simulink model "D_20231120_Modell_Inbetriebnahme_BreakOutBox_Jetson"  (R2022b)
settings: Solver=ode1  StartTime=0.0  StopTime=inf  FixedStep=Ts  RelTol=1e-3
PreLoadFcn:
  | pulsePeriod = 0.05;
  | 
  | Ts = 0.001;
  | 
  | FPGA_Frequency = 75000000;
  | 
  | ts_IO691 = 5e-3;
PostLoadFcn:
  | ewolfSetUp
InitFcn:
  | pulsePeriod = 0.05;
  | 
  | Ts = 0.001;
  | 
  | FPGA_Frequency = 75000000;
  | 
  | ts_IO691 = 5e-3;
StopFcn:
  | Simulink.sdi.clearPreferences;
  | if isfile(['sdi_view_',bdroot,'.mldatx'])
  | Simulink.sdi.view;
  | pause(3);
  | Simulink.sdi.loadView(['sdi_view_',bdroot,]);
  | end
model workspace (MAT data in the model file):
  MaxDreh = 1
values from neighbouring files (symbols this model uses):
  max_ac = 2    [ewolfSetUp.m]
  min_ac = -3    [ewolfSetUp.m]
  PredictionHorizon = 30    [ewolfSetUp.m]
undefined symbols (not defined in the file or in its folder): canChannel, DiscIntNeverNeededParam, Ended, HS, IO291, IO397, max_steer_car, min_steer_car, sigbuilder_block, Single
libraries: lllalib x255, canmsglib x146, simulink x42, speedgoatlib_IO191 x5, speedgoatlib_IO291 x5, slrealtimeiplib x3, speedgoatlib_IO691 x3, slrealtimeutilitieslib x2, spsEdgeDetectorLib x1, simulink_extras x1, speedgoatlib_fpga_dio x1, speedgoatlib_fpga_quadrature x1
(part 4 of 8)

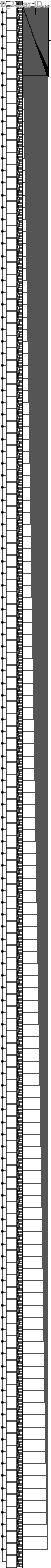
== system D_20231120_Modell_Inbetriebnahme_BreakOutBox_Jetson/IO691/CAN Read Loop - Port 3/Radar IDs einlesen (128) ==
  CAN Msg : Inport
  Bus Creator : BusCreator  Inputs=5
  Bus Creator1 : BusCreator  Inputs=129
  Bus Creator{2..129} (128 alike) : BusCreator  Inputs=8
  CAN Unpack1 : canmsglib/CAN Unpack  CANdbFile=eWolf_SensorCAN.dbc  MsgList=Radar_Sensor_Control  MsgName=Radar_Sensor_Control  MsgIDType=Standard (11-bit identifier)  MsgIdentifier=1024  MsgLength=8  SignalInfo={'Cycle_Duration','0','12','LE','unsigned','Standard','0','0.064','0','0','262';'Cycle_counter','15','32','LE','unsigned','Standard','0','1','0','-Inf','Inf';'Number_of_Objects','47','8','LE','unsigned','Standard','0','1','0','0','255';'Reserve','12','3','LE','unsigned','Standard','0','1','0','-Inf','Inf';'Reserve_2','55','9','LE','unsigned','Standard','0','1','0','-Inf','Inf'}  IDPort=on  TimestampPort=on  ErrorPort=off  RemotePort=off  LengthPort=off  StatusPort=off  ApplyMinMax=off
      settings: DataFormat=CANdb specified signals
  CAN Unpack10 : canmsglib/CAN Unpack  CANdbFile=eWolf_SensorCAN.dbc  MsgList=Radar_RawTarget_Data_009  MsgName=Radar_RawTarget_Data_009  MsgIDType=Standard (11-bit identifier)  MsgIdentifier=1033  MsgLength=8  SignalInfo={'AZ_Winkel','22','10','LE','unsigned','Multiplexed','0','0.16','-81.76','-81.76','81.92';'EL_Angle','37','10','LE','unsigned','Multiplexed','1','0.04','-20.44','-20.44','20.48';'Internal_used','14','8','LE','unsigned','Multiplexed','0','1','0','-Inf','Inf';'Internal_used2','32','7','LE','unsigned','Multiplexed','0','1','0','-Inf','Inf';'Internal_used3','51','7','LE','unsigned','Multiplexed','0','1','0','-Inf','Inf';'Internal_used4','58','6','LE','unsigned','Multiplexed','0','1','0','-Inf','Inf';'Internal_used5','9','8','LE','unsigned','Multiplexed','1','1','0','-Inf','Inf';'Internal_used6','17','8','LE','unsigned','Multiplexed','1','1','0','-Inf','Inf';'Internal_used7','25','7','LE','unsigned','Multiplexed','1','1','0','-Inf','Inf';'Mode_Signal','0','1','LE','unsigned','Multiplexor','0','1','0','0','1';'RCS','1','7','LE','unsigned','Multiplexed','1','0.2','-15','-15','36';'Range1','1','13','LE','unsigned','Multiplexed','0','0.04','0','0','327.64';'Reserve_3','32','5','LE','unsigned','Multiplexed','1','1','0','-Inf','Inf';'Reserve_4','47','16','LE','unsigned','Multiplexed','1','1','0','-Inf','Inf';'Speed_Radial','39','12','LE','unsigned','Multiplexed','0','0.04','-119.68','-44.12','119.68'}  IDPort=on  TimestampPort=on  ErrorPort=off  RemotePort=off  LengthPort=off  StatusPort=off  ApplyMinMax=off
      settings: DataFormat=CANdb specified signals
  CAN Unpack100 : canmsglib/CAN Unpack  CANdbFile=eWolf_SensorCAN.dbc  MsgList=Radar_RawTarget_Data_099  MsgName=Radar_RawTarget_Data_099  MsgIDType=Standard (11-bit identifier)  MsgIdentifier=1123  MsgLength=8  SignalInfo={'AZ_Winkel','22','10','LE','unsigned','Multiplexed','0','0.16','-81.76','-81.76','81.92';'EL_Angle','37','10','LE','unsigned','Multiplexed','1','0.04','-20.44','-20.44','20.48';'Internal_used','14','8','LE','unsigned','Multiplexed','0','1','0','-Inf','Inf';'Internal_used2','32','7','LE','unsigned','Multiplexed','0','1','0','-Inf','Inf';'Internal_used3','51','7','LE','unsigned','Multiplexed','0','1','0','-Inf','Inf';'Internal_used4','58','6','LE','unsigned','Multiplexed','0','1','0','-Inf','Inf';'Internal_used5','9','8','LE','unsigned','Multiplexed','1','1','0','-Inf','Inf';'Internal_used6','17','8','LE','unsigned','Multiplexed','1','1','0','-Inf','Inf';'Internal_used7','25','7','LE','unsigned','Multiplexed','1','1','0','-Inf','Inf';'Mode_Signal','0','1','LE','unsigned','Multiplexor','0','1','0','0','1';'RCS','1','7','LE','unsigned','Multiplexed','1','0.2','-15','-15','36';'Range1','1','13','LE','unsigned','Multiplexed','0','0.04','0','0','327.64';'Reserve_3','32','5','LE','unsigned','Multiplexed','1','1','0','-Inf','Inf';'Reserve_4','47','16','LE','unsigned','Multiplexed','1','1','0','-Inf','Inf';'Speed_Radial','39','12','LE','unsigned','Multiplexed','0','0.04','-119.68','-44.12','119.68'}  IDPort=on  TimestampPort=on  ErrorPort=off  RemotePort=off  LengthPort=off  StatusPort=off  ApplyMinMax=off
      settings: DataFormat=CANdb specified signals
  CAN Unpack101 : canmsglib/CAN Unpack  CANdbFile=eWolf_SensorCAN.dbc  MsgList=Radar_RawTarget_Data_100  MsgName=Radar_RawTarget_Data_100  MsgIDType=Standard (11-bit identifier)  MsgIdentifier=1124  MsgLength=8  SignalInfo={'AZ_Winkel','22','10','LE','unsigned','Multiplexed','0','0.16','-81.76','-81.76','81.92';'EL_Angle','37','10','LE','unsigned','Multiplexed','1','0.04','-20.44','-20.44','20.48';'Internal_used','14','8','LE','unsigned','Multiplexed','0','1','0','-Inf','Inf';'Internal_used2','32','7','LE','unsigned','Multiplexed','0','1','0','-Inf','Inf';'Internal_used3','51','7','LE','unsigned','Multiplexed','0','1','0','-Inf','Inf';'Internal_used4','58','6','LE','unsigned','Multiplexed','0','1','0','-Inf','Inf';'Internal_used5','9','8','LE','unsigned','Multiplexed','1','1','0','-Inf','Inf';'Internal_used6','17','8','LE','unsigned','Multiplexed','1','1','0','-Inf','Inf';'Internal_used7','25','7','LE','unsigned','Multiplexed','1','1','0','-Inf','Inf';'Mode_Signal','0','1','LE','unsigned','Multiplexor','0','1','0','0','1';'RCS','1','7','LE','unsigned','Multiplexed','1','0.2','-15','-15','36';'Range1','1','13','LE','unsigned','Multiplexed','0','0.04','0','0','327.64';'Reserve_3','32','5','LE','unsigned','Multiplexed','1','1','0','-Inf','Inf';'Reserve_4','47','16','LE','unsigned','Multiplexed','1','1','0','-Inf','Inf';'Speed_Radial','39','12','LE','unsigned','Multiplexed','0','0.04','-119.68','-44.12','119.68'}  IDPort=on  TimestampPort=on  ErrorPort=off  RemotePort=off  LengthPort=off  StatusPort=off  ApplyMinMax=off
      settings: DataFormat=CANdb specified signals
  CAN Unpack102 : canmsglib/CAN Unpack  CANdbFile=eWolf_SensorCAN.dbc  MsgList=Radar_RawTarget_Data_101  MsgName=Radar_RawTarget_Data_101  MsgIDType=Standard (11-bit identifier)  MsgIdentifier=1125  MsgLength=8  SignalInfo={'AZ_Winkel','22','10','LE','unsigned','Multiplexed','0','0.16','-81.76','-81.76','81.92';'EL_Angle','37','10','LE','unsigned','Multiplexed','1','0.04','-20.44','-20.44','20.48';'Internal_used','14','8','LE','unsigned','Multiplexed','0','1','0','-Inf','Inf';'Internal_used2','32','7','LE','unsigned','Multiplexed','0','1','0','-Inf','Inf';'Internal_used3','51','7','LE','unsigned','Multiplexed','0','1','0','-Inf','Inf';'Internal_used4','58','6','LE','unsigned','Multiplexed','0','1','0','-Inf','Inf';'Internal_used5','9','8','LE','unsigned','Multiplexed','1','1','0','-Inf','Inf';'Internal_used6','17','8','LE','unsigned','Multiplexed','1','1','0','-Inf','Inf';'Internal_used7','25','7','LE','unsigned','Multiplexed','1','1','0','-Inf','Inf';'Mode_Signal','0','1','LE','unsigned','Multiplexor','0','1','0','0','1';'RCS','1','7','LE','unsigned','Multiplexed','1','0.2','-15','-15','36';'Range1','1','13','LE','unsigned','Multiplexed','0','0.04','0','0','327.64';'Reserve_3','32','5','LE','unsigned','Multiplexed','1','1','0','-Inf','Inf';'Reserve_4','47','16','LE','unsigned','Multiplexed','1','1','0','-Inf','Inf';'Speed_Radial','39','12','LE','unsigned','Multiplexed','0','0.04','-119.68','-44.12','119.68'}  IDPort=on  TimestampPort=on  ErrorPort=off  RemotePort=off  LengthPort=off  StatusPort=off  ApplyMinMax=off
      settings: DataFormat=CANdb specified signals
  CAN Unpack103 : canmsglib/CAN Unpack  CANdbFile=eWolf_SensorCAN.dbc  MsgList=Radar_RawTarget_Data_102  MsgName=Radar_RawTarget_Data_102  MsgIDType=Standard (11-bit identifier)  MsgIdentifier=1126  MsgLength=8  SignalInfo={'AZ_Winkel','22','10','LE','unsigned','Multiplexed','0','0.16','-81.76','-81.76','81.92';'EL_Angle','37','10','LE','unsigned','Multiplexed','1','0.04','-20.44','-20.44','20.48';'Internal_used','14','8','LE','unsigned','Multiplexed','0','1','0','-Inf','Inf';'Internal_used2','32','7','LE','unsigned','Multiplexed','0','1','0','-Inf','Inf';'Internal_used3','51','7','LE','unsigned','Multiplexed','0','1','0','-Inf','Inf';'Internal_used4','58','6','LE','unsigned','Multiplexed','0','1','0','-Inf','Inf';'Internal_used5','9','8','LE','unsigned','Multiplexed','1','1','0','-Inf','Inf';'Internal_used6','17','8','LE','unsigned','Multiplexed','1','1','0','-Inf','Inf';'Internal_used7','25','7','LE','unsigned','Multiplexed','1','1','0','-Inf','Inf';'Mode_Signal','0','1','LE','unsigned','Multiplexor','0','1','0','0','1';'RCS','1','7','LE','unsigned','Multiplexed','1','0.2','-15','-15','36';'Range1','1','13','LE','unsigned','Multiplexed','0','0.04','0','0','327.64';'Reserve_3','32','5','LE','unsigned','Multiplexed','1','1','0','-Inf','Inf';'Reserve_4','47','16','LE','unsigned','Multiplexed','1','1','0','-Inf','Inf';'Speed_Radial','39','12','LE','unsigned','Multiplexed','0','0.04','-119.68','-44.12','119.68'}  IDPort=on  TimestampPort=on  ErrorPort=off  RemotePort=off  LengthPort=off  StatusPort=off  ApplyMinMax=off
      settings: DataFormat=CANdb specified signals
  CAN Unpack104 : canmsglib/CAN Unpack  CANdbFile=eWolf_SensorCAN.dbc  MsgList=Radar_RawTarget_Data_103  MsgName=Radar_RawTarget_Data_103  MsgIDType=Standard (11-bit identifier)  MsgIdentifier=1127  MsgLength=8  SignalInfo={'AZ_Winkel','22','10','LE','unsigned','Multiplexed','0','0.16','-81.76','-81.76','81.92';'EL_Angle','37','10','LE','unsigned','Multiplexed','1','0.04','-20.44','-20.44','20.48';'Internal_used','14','8','LE','unsigned','Multiplexed','0','1','0','-Inf','Inf';'Internal_used2','32','7','LE','unsigned','Multiplexed','0','1','0','-Inf','Inf';'Internal_used3','51','7','LE','unsigned','Multiplexed','0','1','0','-Inf','Inf';'Internal_used4','58','6','LE','unsigned','Multiplexed','0','1','0','-Inf','Inf';'Internal_used5','9','8','LE','unsigned','Multiplexed','1','1','0','-Inf','Inf';'Internal_used6','17','8','LE','unsigned','Multiplexed','1','1','0','-Inf','Inf';'Internal_used7','25','7','LE','unsigned','Multiplexed','1','1','0','-Inf','Inf';'Mode_Signal','0','1','LE','unsigned','Multiplexor','0','1','0','0','1';'RCS','1','7','LE','unsigned','Multiplexed','1','0.2','-15','-15','36';'Range1','1','13','LE','unsigned','Multiplexed','0','0.04','0','0','327.64';'Reserve_3','32','5','LE','unsigned','Multiplexed','1','1','0','-Inf','Inf';'Reserve_4','47','16','LE','unsigned','Multiplexed','1','1','0','-Inf','Inf';'Speed_Radial','39','12','LE','unsigned','Multiplexed','0','0.04','-119.68','-44.12','119.68'}  IDPort=on  TimestampPort=on  ErrorPort=off  RemotePort=off  LengthPort=off  StatusPort=off  ApplyMinMax=off
      settings: DataFormat=CANdb specified signals
  CAN Unpack105 : canmsglib/CAN Unpack  CANdbFile=eWolf_SensorCAN.dbc  MsgList=Radar_RawTarget_Data_104  MsgName=Radar_RawTarget_Data_104  MsgIDType=Standard (11-bit identifier)  MsgIdentifier=1128  MsgLength=8  SignalInfo={'AZ_Winkel','22','10','LE','unsigned','Multiplexed','0','0.16','-81.76','-81.76','81.92';'EL_Angle','37','10','LE','unsigned','Multiplexed','1','0.04','-20.44','-20.44','20.48';'Internal_used','14','8','LE','unsigned','Multiplexed','0','1','0','-Inf','Inf';'Internal_used2','32','7','LE','unsigned','Multiplexed','0','1','0','-Inf','Inf';'Internal_used3','51','7','LE','unsigned','Multiplexed','0','1','0','-Inf','Inf';'Internal_used4','58','6','LE','unsigned','Multiplexed','0','1','0','-Inf','Inf';'Internal_used5','9','8','LE','unsigned','Multiplexed','1','1','0','-Inf','Inf';'Internal_used6','17','8','LE','unsigned','Multiplexed','1','1','0','-Inf','Inf';'Internal_used7','25','7','LE','unsigned','Multiplexed','1','1','0','-Inf','Inf';'Mode_Signal','0','1','LE','unsigned','Multiplexor','0','1','0','0','1';'RCS','1','7','LE','unsigned','Multiplexed','1','0.2','-15','-15','36';'Range1','1','13','LE','unsigned','Multiplexed','0','0.04','0','0','327.64';'Reserve_3','32','5','LE','unsigned','Multiplexed','1','1','0','-Inf','Inf';'Reserve_4','47','16','LE','unsigned','Multiplexed','1','1','0','-Inf','Inf';'Speed_Radial','39','12','LE','unsigned','Multiplexed','0','0.04','-119.68','-44.12','119.68'}  IDPort=on  TimestampPort=on  ErrorPort=off  RemotePort=off  LengthPort=off  StatusPort=off  ApplyMinMax=off
      settings: DataFormat=CANdb specified signals
  CAN Unpack106 : canmsglib/CAN Unpack  CANdbFile=eWolf_SensorCAN.dbc  MsgList=Radar_RawTarget_Data_105  MsgName=Radar_RawTarget_Data_105  MsgIDType=Standard (11-bit identifier)  MsgIdentifier=1129  MsgLength=8  SignalInfo={'AZ_Winkel','22','10','LE','unsigned','Multiplexed','0','0.16','-81.76','-81.76','81.92';'EL_Angle','37','10','LE','unsigned','Multiplexed','1','0.04','-20.44','-20.44','20.48';'Internal_used','14','8','LE','unsigned','Multiplexed','0','1','0','-Inf','Inf';'Internal_used2','32','7','LE','unsigned','Multiplexed','0','1','0','-Inf','Inf';'Internal_used3','51','7','LE','unsigned','Multiplexed','0','1','0','-Inf','Inf';'Internal_used4','58','6','LE','unsigned','Multiplexed','0','1','0','-Inf','Inf';'Internal_used5','9','8','LE','unsigned','Multiplexed','1','1','0','-Inf','Inf';'Internal_used6','17','8','LE','unsigned','Multiplexed','1','1','0','-Inf','Inf';'Internal_used7','25','7','LE','unsigned','Multiplexed','1','1','0','-Inf','Inf';'Mode_Signal','0','1','LE','unsigned','Multiplexor','0','1','0','0','1';'RCS','1','7','LE','unsigned','Multiplexed','1','0.2','-15','-15','36';'Range1','1','13','LE','unsigned','Multiplexed','0','0.04','0','0','327.64';'Reserve_3','32','5','LE','unsigned','Multiplexed','1','1','0','-Inf','Inf';'Reserve_4','47','16','LE','unsigned','Multiplexed','1','1','0','-Inf','Inf';'Speed_Radial','39','12','LE','unsigned','Multiplexed','0','0.04','-119.68','-44.12','119.68'}  IDPort=on  TimestampPort=on  ErrorPort=off  RemotePort=off  LengthPort=off  StatusPort=off  ApplyMinMax=off
      settings: DataFormat=CANdb specified signals
  CAN Unpack107 : canmsglib/CAN Unpack  CANdbFile=eWolf_SensorCAN.dbc  MsgList=Radar_RawTarget_Data_106  MsgName=Radar_RawTarget_Data_106  MsgIDType=Standard (11-bit identifier)  MsgIdentifier=1130  MsgLength=8  SignalInfo={'AZ_Winkel','22','10','LE','unsigned','Multiplexed','0','0.16','-81.76','-81.76','81.92';'EL_Angle','37','10','LE','unsigned','Multiplexed','1','0.04','-20.44','-20.44','20.48';'Internal_used','14','8','LE','unsigned','Multiplexed','0','1','0','-Inf','Inf';'Internal_used2','32','7','LE','unsigned','Multiplexed','0','1','0','-Inf','Inf';'Internal_used3','51','7','LE','unsigned','Multiplexed','0','1','0','-Inf','Inf';'Internal_used4','58','6','LE','unsigned','Multiplexed','0','1','0','-Inf','Inf';'Internal_used5','9','8','LE','unsigned','Multiplexed','1','1','0','-Inf','Inf';'Internal_used6','17','8','LE','unsigned','Multiplexed','1','1','0','-Inf','Inf';'Internal_used7','25','7','LE','unsigned','Multiplexed','1','1','0','-Inf','Inf';'Mode_Signal','0','1','LE','unsigned','Multiplexor','0','1','0','0','1';'RCS','1','7','LE','unsigned','Multiplexed','1','0.2','-15','-15','36';'Range1','1','13','LE','unsigned','Multiplexed','0','0.04','0','0','327.64';'Reserve_3','32','5','LE','unsigned','Multiplexed','1','1','0','-Inf','Inf';'Reserve_4','47','16','LE','unsigned','Multiplexed','1','1','0','-Inf','Inf';'Speed_Radial','39','12','LE','unsigned','Multiplexed','0','0.04','-119.68','-44.12','119.68'}  IDPort=on  TimestampPort=on  ErrorPort=off  RemotePort=off  LengthPort=off  StatusPort=off  ApplyMinMax=off
      settings: DataFormat=CANdb specified signals
  CAN Unpack108 : canmsglib/CAN Unpack  CANdbFile=eWolf_SensorCAN.dbc  MsgList=Radar_RawTarget_Data_107  MsgName=Radar_RawTarget_Data_107  MsgIDType=Standard (11-bit identifier)  MsgIdentifier=1131  MsgLength=8  SignalInfo={'AZ_Winkel','22','10','LE','unsigned','Multiplexed','0','0.16','-81.76','-81.76','81.92';'EL_Angle','37','10','LE','unsigned','Multiplexed','1','0.04','-20.44','-20.44','20.48';'Internal_used','14','8','LE','unsigned','Multiplexed','0','1','0','-Inf','Inf';'Internal_used2','32','7','LE','unsigned','Multiplexed','0','1','0','-Inf','Inf';'Internal_used3','51','7','LE','unsigned','Multiplexed','0','1','0','-Inf','Inf';'Internal_used4','58','6','LE','unsigned','Multiplexed','0','1','0','-Inf','Inf';'Internal_used5','9','8','LE','unsigned','Multiplexed','1','1','0','-Inf','Inf';'Internal_used6','17','8','LE','unsigned','Multiplexed','1','1','0','-Inf','Inf';'Internal_used7','25','7','LE','unsigned','Multiplexed','1','1','0','-Inf','Inf';'Mode_Signal','0','1','LE','unsigned','Multiplexor','0','1','0','0','1';'RCS','1','7','LE','unsigned','Multiplexed','1','0.2','-15','-15','36';'Range1','1','13','LE','unsigned','Multiplexed','0','0.04','0','0','327.64';'Reserve_3','32','5','LE','unsigned','Multiplexed','1','1','0','-Inf','Inf';'Reserve_4','47','16','LE','unsigned','Multiplexed','1','1','0','-Inf','Inf';'Speed_Radial','39','12','LE','unsigned','Multiplexed','0','0.04','-119.68','-44.12','119.68'}  IDPort=on  TimestampPort=on  ErrorPort=off  RemotePort=off  LengthPort=off  StatusPort=off  ApplyMinMax=off
      settings: DataFormat=CANdb specified signals
  CAN Unpack109 : canmsglib/CAN Unpack  CANdbFile=eWolf_SensorCAN.dbc  MsgList=Radar_RawTarget_Data_108  MsgName=Radar_RawTarget_Data_108  MsgIDType=Standard (11-bit identifier)  MsgIdentifier=1132  MsgLength=8  SignalInfo={'AZ_Winkel','22','10','LE','unsigned','Multiplexed','0','0.16','-81.76','-81.76','81.92';'EL_Angle','37','10','LE','unsigned','Multiplexed','1','0.04','-20.44','-20.44','20.48';'Internal_used','14','8','LE','unsigned','Multiplexed','0','1','0','-Inf','Inf';'Internal_used2','32','7','LE','unsigned','Multiplexed','0','1','0','-Inf','Inf';'Internal_used3','51','7','LE','unsigned','Multiplexed','0','1','0','-Inf','Inf';'Internal_used4','58','6','LE','unsigned','Multiplexed','0','1','0','-Inf','Inf';'Internal_used5','9','8','LE','unsigned','Multiplexed','1','1','0','-Inf','Inf';'Internal_used6','17','8','LE','unsigned','Multiplexed','1','1','0','-Inf','Inf';'Internal_used7','25','7','LE','unsigned','Multiplexed','1','1','0','-Inf','Inf';'Mode_Signal','0','1','LE','unsigned','Multiplexor','0','1','0','0','1';'RCS','1','7','LE','unsigned','Multiplexed','1','0.2','-15','-15','36';'Range1','1','13','LE','unsigned','Multiplexed','0','0.04','0','0','327.64';'Reserve_3','32','5','LE','unsigned','Multiplexed','1','1','0','-Inf','Inf';'Reserve_4','47','16','LE','unsigned','Multiplexed','1','1','0','-Inf','Inf';'Speed_Radial','39','12','LE','unsigned','Multiplexed','0','0.04','-119.68','-44.12','119.68'}  IDPort=on  TimestampPort=on  ErrorPort=off  RemotePort=off  LengthPort=off  StatusPort=off  ApplyMinMax=off
      settings: DataFormat=CANdb specified signals
  CAN Unpack11 : canmsglib/CAN Unpack  CANdbFile=eWolf_SensorCAN.dbc  MsgList=Radar_RawTarget_Data_010  MsgName=Radar_RawTarget_Data_010  MsgIDType=Standard (11-bit identifier)  MsgIdentifier=1034  MsgLength=8  SignalInfo={'AZ_Winkel','22','10','LE','unsigned','Multiplexed','0','0.16','-81.76','-81.76','81.92';'EL_Angle','37','10','LE','unsigned','Multiplexed','1','0.04','-20.44','-20.44','20.48';'Internal_used','14','8','LE','unsigned','Multiplexed','0','1','0','-Inf','Inf';'Internal_used2','32','7','LE','unsigned','Multiplexed','0','1','0','-Inf','Inf';'Internal_used3','51','7','LE','unsigned','Multiplexed','0','1','0','-Inf','Inf';'Internal_used4','58','6','LE','unsigned','Multiplexed','0','1','0','-Inf','Inf';'Internal_used5','9','8','LE','unsigned','Multiplexed','1','1','0','-Inf','Inf';'Internal_used6','17','8','LE','unsigned','Multiplexed','1','1','0','-Inf','Inf';'Internal_used7','25','7','LE','unsigned','Multiplexed','1','1','0','-Inf','Inf';'Mode_Signal','0','1','LE','unsigned','Multiplexor','0','1','0','0','1';'RCS','1','7','LE','unsigned','Multiplexed','1','0.2','-15','-15','36';'Range1','1','13','LE','unsigned','Multiplexed','0','0.04','0','0','327.64';'Reserve_3','32','5','LE','unsigned','Multiplexed','1','1','0','-Inf','Inf';'Reserve_4','47','16','LE','unsigned','Multiplexed','1','1','0','-Inf','Inf';'Speed_Radial','39','12','LE','unsigned','Multiplexed','0','0.04','-119.68','-44.12','119.68'}  IDPort=on  TimestampPort=on  ErrorPort=off  RemotePort=off  LengthPort=off  StatusPort=off  ApplyMinMax=off
      settings: DataFormat=CANdb specified signals
  CAN Unpack110 : canmsglib/CAN Unpack  CANdbFile=eWolf_SensorCAN.dbc  MsgList=Radar_RawTarget_Data_109  MsgName=Radar_RawTarget_Data_109  MsgIDType=Standard (11-bit identifier)  MsgIdentifier=1133  MsgLength=8  SignalInfo={'AZ_Winkel','22','10','LE','unsigned','Multiplexed','0','0.16','-81.76','-81.76','81.92';'EL_Angle','37','10','LE','unsigned','Multiplexed','1','0.04','-20.44','-20.44','20.48';'Internal_used','14','8','LE','unsigned','Multiplexed','0','1','0','-Inf','Inf';'Internal_used2','32','7','LE','unsigned','Multiplexed','0','1','0','-Inf','Inf';'Internal_used3','51','7','LE','unsigned','Multiplexed','0','1','0','-Inf','Inf';'Internal_used4','58','6','LE','unsigned','Multiplexed','0','1','0','-Inf','Inf';'Internal_used5','9','8','LE','unsigned','Multiplexed','1','1','0','-Inf','Inf';'Internal_used6','17','8','LE','unsigned','Multiplexed','1','1','0','-Inf','Inf';'Internal_used7','25','7','LE','unsigned','Multiplexed','1','1','0','-Inf','Inf';'Mode_Signal','0','1','LE','unsigned','Multiplexor','0','1','0','0','1';'RCS','1','7','LE','unsigned','Multiplexed','1','0.2','-15','-15','36';'Range1','1','13','LE','unsigned','Multiplexed','0','0.04','0','0','327.64';'Reserve_3','32','5','LE','unsigned','Multiplexed','1','1','0','-Inf','Inf';'Reserve_4','47','16','LE','unsigned','Multiplexed','1','1','0','-Inf','Inf';'Speed_Radial','39','12','LE','unsigned','Multiplexed','0','0.04','-119.68','-44.12','119.68'}  IDPort=on  TimestampPort=on  ErrorPort=off  RemotePort=off  LengthPort=off  StatusPort=off  ApplyMinMax=off
      settings: DataFormat=CANdb specified signals
  CAN Unpack111 : canmsglib/CAN Unpack  CANdbFile=eWolf_SensorCAN.dbc  MsgList=Radar_RawTarget_Data_110  MsgName=Radar_RawTarget_Data_110  MsgIDType=Standard (11-bit identifier)  MsgIdentifier=1134  MsgLength=8  SignalInfo={'AZ_Winkel','22','10','LE','unsigned','Multiplexed','0','0.16','-81.76','-81.76','81.92';'EL_Angle','37','10','LE','unsigned','Multiplexed','1','0.04','-20.44','-20.44','20.48';'Internal_used','14','8','LE','unsigned','Multiplexed','0','1','0','-Inf','Inf';'Internal_used2','32','7','LE','unsigned','Multiplexed','0','1','0','-Inf','Inf';'Internal_used3','51','7','LE','unsigned','Multiplexed','0','1','0','-Inf','Inf';'Internal_used4','58','6','LE','unsigned','Multiplexed','0','1','0','-Inf','Inf';'Internal_used5','9','8','LE','unsigned','Multiplexed','1','1','0','-Inf','Inf';'Internal_used6','17','8','LE','unsigned','Multiplexed','1','1','0','-Inf','Inf';'Internal_used7','25','7','LE','unsigned','Multiplexed','1','1','0','-Inf','Inf';'Mode_Signal','0','1','LE','unsigned','Multiplexor','0','1','0','0','1';'RCS','1','7','LE','unsigned','Multiplexed','1','0.2','-15','-15','36';'Range1','1','13','LE','unsigned','Multiplexed','0','0.04','0','0','327.64';'Reserve_3','32','5','LE','unsigned','Multiplexed','1','1','0','-Inf','Inf';'Reserve_4','47','16','LE','unsigned','Multiplexed','1','1','0','-Inf','Inf';'Speed_Radial','39','12','LE','unsigned','Multiplexed','0','0.04','-119.68','-44.12','119.68'}  IDPort=on  TimestampPort=on  ErrorPort=off  RemotePort=off  LengthPort=off  StatusPort=off  ApplyMinMax=off
      settings: DataFormat=CANdb specified signals
  CAN Unpack112 : canmsglib/CAN Unpack  CANdbFile=eWolf_SensorCAN.dbc  MsgList=Radar_RawTarget_Data_111  MsgName=Radar_RawTarget_Data_111  MsgIDType=Standard (11-bit identifier)  MsgIdentifier=1135  MsgLength=8  SignalInfo={'AZ_Winkel','22','10','LE','unsigned','Multiplexed','0','0.16','-81.76','-81.76','81.92';'EL_Angle','37','10','LE','unsigned','Multiplexed','1','0.04','-20.44','-20.44','20.48';'Internal_used','14','8','LE','unsigned','Multiplexed','0','1','0','-Inf','Inf';'Internal_used2','32','7','LE','unsigned','Multiplexed','0','1','0','-Inf','Inf';'Internal_used3','51','7','LE','unsigned','Multiplexed','0','1','0','-Inf','Inf';'Internal_used4','58','6','LE','unsigned','Multiplexed','0','1','0','-Inf','Inf';'Internal_used5','9','8','LE','unsigned','Multiplexed','1','1','0','-Inf','Inf';'Internal_used6','17','8','LE','unsigned','Multiplexed','1','1','0','-Inf','Inf';'Internal_used7','25','7','LE','unsigned','Multiplexed','1','1','0','-Inf','Inf';'Mode_Signal','0','1','LE','unsigned','Multiplexor','0','1','0','0','1';'RCS','1','7','LE','unsigned','Multiplexed','1','0.2','-15','-15','36';'Range1','1','13','LE','unsigned','Multiplexed','0','0.04','0','0','327.64';'Reserve_3','32','5','LE','unsigned','Multiplexed','1','1','0','-Inf','Inf';'Reserve_4','47','16','LE','unsigned','Multiplexed','1','1','0','-Inf','Inf';'Speed_Radial','39','12','LE','unsigned','Multiplexed','0','0.04','-119.68','-44.12','119.68'}  IDPort=on  TimestampPort=on  ErrorPort=off  RemotePort=off  LengthPort=off  StatusPort=off  ApplyMinMax=off
      settings: DataFormat=CANdb specified signals
  CAN Unpack113 : canmsglib/CAN Unpack  CANdbFile=eWolf_SensorCAN.dbc  MsgList=Radar_RawTarget_Data_112  MsgName=Radar_RawTarget_Data_112  MsgIDType=Standard (11-bit identifier)  MsgIdentifier=1136  MsgLength=8  SignalInfo={'AZ_Winkel','22','10','LE','unsigned','Multiplexed','0','0.16','-81.76','-81.76','81.92';'EL_Angle','37','10','LE','unsigned','Multiplexed','1','0.04','-20.44','-20.44','20.48';'Internal_used','14','8','LE','unsigned','Multiplexed','0','1','0','-Inf','Inf';'Internal_used2','32','7','LE','unsigned','Multiplexed','0','1','0','-Inf','Inf';'Internal_used3','51','7','LE','unsigned','Multiplexed','0','1','0','-Inf','Inf';'Internal_used4','58','6','LE','unsigned','Multiplexed','0','1','0','-Inf','Inf';'Internal_used5','9','8','LE','unsigned','Multiplexed','1','1','0','-Inf','Inf';'Internal_used6','17','8','LE','unsigned','Multiplexed','1','1','0','-Inf','Inf';'Internal_used7','25','7','LE','unsigned','Multiplexed','1','1','0','-Inf','Inf';'Mode_Signal','0','1','LE','unsigned','Multiplexor','0','1','0','0','1';'RCS','1','7','LE','unsigned','Multiplexed','1','0.2','-15','-15','36';'Range1','1','13','LE','unsigned','Multiplexed','0','0.04','0','0','327.64';'Reserve_3','32','5','LE','unsigned','Multiplexed','1','1','0','-Inf','Inf';'Reserve_4','47','16','LE','unsigned','Multiplexed','1','1','0','-Inf','Inf';'Speed_Radial','39','12','LE','unsigned','Multiplexed','0','0.04','-119.68','-44.12','119.68'}  IDPort=on  TimestampPort=on  ErrorPort=off  RemotePort=off  LengthPort=off  StatusPort=off  ApplyMinMax=off
      settings: DataFormat=CANdb specified signals
  CAN Unpack114 : canmsglib/CAN Unpack  CANdbFile=eWolf_SensorCAN.dbc  MsgList=Radar_RawTarget_Data_113  MsgName=Radar_RawTarget_Data_113  MsgIDType=Standard (11-bit identifier)  MsgIdentifier=1137  MsgLength=8  SignalInfo={'AZ_Winkel','22','10','LE','unsigned','Multiplexed','0','0.16','-81.76','-81.76','81.92';'EL_Angle','37','10','LE','unsigned','Multiplexed','1','0.04','-20.44','-20.44','20.48';'Internal_used','14','8','LE','unsigned','Multiplexed','0','1','0','-Inf','Inf';'Internal_used2','32','7','LE','unsigned','Multiplexed','0','1','0','-Inf','Inf';'Internal_used3','51','7','LE','unsigned','Multiplexed','0','1','0','-Inf','Inf';'Internal_used4','58','6','LE','unsigned','Multiplexed','0','1','0','-Inf','Inf';'Internal_used5','9','8','LE','unsigned','Multiplexed','1','1','0','-Inf','Inf';'Internal_used6','17','8','LE','unsigned','Multiplexed','1','1','0','-Inf','Inf';'Internal_used7','25','7','LE','unsigned','Multiplexed','1','1','0','-Inf','Inf';'Mode_Signal','0','1','LE','unsigned','Multiplexor','0','1','0','0','1';'RCS','1','7','LE','unsigned','Multiplexed','1','0.2','-15','-15','36';'Range1','1','13','LE','unsigned','Multiplexed','0','0.04','0','0','327.64';'Reserve_3','32','5','LE','unsigned','Multiplexed','1','1','0','-Inf','Inf';'Reserve_4','47','16','LE','unsigned','Multiplexed','1','1','0','-Inf','Inf';'Speed_Radial','39','12','LE','unsigned','Multiplexed','0','0.04','-119.68','-44.12','119.68'}  IDPort=on  TimestampPort=on  ErrorPort=off  RemotePort=off  LengthPort=off  StatusPort=off  ApplyMinMax=off
      settings: DataFormat=CANdb specified signals
  CAN Unpack115 : canmsglib/CAN Unpack  CANdbFile=eWolf_SensorCAN.dbc  MsgList=Radar_RawTarget_Data_114  MsgName=Radar_RawTarget_Data_114  MsgIDType=Standard (11-bit identifier)  MsgIdentifier=1138  MsgLength=8  SignalInfo={'AZ_Winkel','22','10','LE','unsigned','Multiplexed','0','0.16','-81.76','-81.76','81.92';'EL_Angle','37','10','LE','unsigned','Multiplexed','1','0.04','-20.44','-20.44','20.48';'Internal_used','14','8','LE','unsigned','Multiplexed','0','1','0','-Inf','Inf';'Internal_used2','32','7','LE','unsigned','Multiplexed','0','1','0','-Inf','Inf';'Internal_used3','51','7','LE','unsigned','Multiplexed','0','1','0','-Inf','Inf';'Internal_used4','58','6','LE','unsigned','Multiplexed','0','1','0','-Inf','Inf';'Internal_used5','9','8','LE','unsigned','Multiplexed','1','1','0','-Inf','Inf';'Internal_used6','17','8','LE','unsigned','Multiplexed','1','1','0','-Inf','Inf';'Internal_used7','25','7','LE','unsigned','Multiplexed','1','1','0','-Inf','Inf';'Mode_Signal','0','1','LE','unsigned','Multiplexor','0','1','0','0','1';'RCS','1','7','LE','unsigned','Multiplexed','1','0.2','-15','-15','36';'Range1','1','13','LE','unsigned','Multiplexed','0','0.04','0','0','327.64';'Reserve_3','32','5','LE','unsigned','Multiplexed','1','1','0','-Inf','Inf';'Reserve_4','47','16','LE','unsigned','Multiplexed','1','1','0','-Inf','Inf';'Speed_Radial','39','12','LE','unsigned','Multiplexed','0','0.04','-119.68','-44.12','119.68'}  IDPort=on  TimestampPort=on  ErrorPort=off  RemotePort=off  LengthPort=off  StatusPort=off  ApplyMinMax=off
      settings: DataFormat=CANdb specified signals
  CAN Unpack116 : canmsglib/CAN Unpack  CANdbFile=eWolf_SensorCAN.dbc  MsgList=Radar_RawTarget_Data_115  MsgName=Radar_RawTarget_Data_115  MsgIDType=Standard (11-bit identifier)  MsgIdentifier=1139  MsgLength=8  SignalInfo={'AZ_Winkel','22','10','LE','unsigned','Multiplexed','0','0.16','-81.76','-81.76','81.92';'EL_Angle','37','10','LE','unsigned','Multiplexed','1','0.04','-20.44','-20.44','20.48';'Internal_used','14','8','LE','unsigned','Multiplexed','0','1','0','-Inf','Inf';'Internal_used2','32','7','LE','unsigned','Multiplexed','0','1','0','-Inf','Inf';'Internal_used3','51','7','LE','unsigned','Multiplexed','0','1','0','-Inf','Inf';'Internal_used4','58','6','LE','unsigned','Multiplexed','0','1','0','-Inf','Inf';'Internal_used5','9','8','LE','unsigned','Multiplexed','1','1','0','-Inf','Inf';'Internal_used6','17','8','LE','unsigned','Multiplexed','1','1','0','-Inf','Inf';'Internal_used7','25','7','LE','unsigned','Multiplexed','1','1','0','-Inf','Inf';'Mode_Signal','0','1','LE','unsigned','Multiplexor','0','1','0','0','1';'RCS','1','7','LE','unsigned','Multiplexed','1','0.2','-15','-15','36';'Range1','1','13','LE','unsigned','Multiplexed','0','0.04','0','0','327.64';'Reserve_3','32','5','LE','unsigned','Multiplexed','1','1','0','-Inf','Inf';'Reserve_4','47','16','LE','unsigned','Multiplexed','1','1','0','-Inf','Inf';'Speed_Radial','39','12','LE','unsigned','Multiplexed','0','0.04','-119.68','-44.12','119.68'}  IDPort=on  TimestampPort=on  ErrorPort=off  RemotePort=off  LengthPort=off  StatusPort=off  ApplyMinMax=off
      settings: DataFormat=CANdb specified signals
  CAN Unpack117 : canmsglib/CAN Unpack  CANdbFile=eWolf_SensorCAN.dbc  MsgList=Radar_RawTarget_Data_116  MsgName=Radar_RawTarget_Data_116  MsgIDType=Standard (11-bit identifier)  MsgIdentifier=1140  MsgLength=8  SignalInfo={'AZ_Winkel','22','10','LE','unsigned','Multiplexed','0','0.16','-81.76','-81.76','81.92';'EL_Angle','37','10','LE','unsigned','Multiplexed','1','0.04','-20.44','-20.44','20.48';'Internal_used','14','8','LE','unsigned','Multiplexed','0','1','0','-Inf','Inf';'Internal_used2','32','7','LE','unsigned','Multiplexed','0','1','0','-Inf','Inf';'Internal_used3','51','7','LE','unsigned','Multiplexed','0','1','0','-Inf','Inf';'Internal_used4','58','6','LE','unsigned','Multiplexed','0','1','0','-Inf','Inf';'Internal_used5','9','8','LE','unsigned','Multiplexed','1','1','0','-Inf','Inf';'Internal_used6','17','8','LE','unsigned','Multiplexed','1','1','0','-Inf','Inf';'Internal_used7','25','7','LE','unsigned','Multiplexed','1','1','0','-Inf','Inf';'Mode_Signal','0','1','LE','unsigned','Multiplexor','0','1','0','0','1';'RCS','1','7','LE','unsigned','Multiplexed','1','0.2','-15','-15','36';'Range1','1','13','LE','unsigned','Multiplexed','0','0.04','0','0','327.64';'Reserve_3','32','5','LE','unsigned','Multiplexed','1','1','0','-Inf','Inf';'Reserve_4','47','16','LE','unsigned','Multiplexed','1','1','0','-Inf','Inf';'Speed_Radial','39','12','LE','unsigned','Multiplexed','0','0.04','-119.68','-44.12','119.68'}  IDPort=on  TimestampPort=on  ErrorPort=off  RemotePort=off  LengthPort=off  StatusPort=off  ApplyMinMax=off
      settings: DataFormat=CANdb specified signals
  CAN Unpack118 : canmsglib/CAN Unpack  CANdbFile=eWolf_SensorCAN.dbc  MsgList=Radar_RawTarget_Data_117  MsgName=Radar_RawTarget_Data_117  MsgIDType=Standard (11-bit identifier)  MsgIdentifier=1141  MsgLength=8  SignalInfo={'AZ_Winkel','22','10','LE','unsigned','Multiplexed','0','0.16','-81.76','-81.76','81.92';'EL_Angle','37','10','LE','unsigned','Multiplexed','1','0.04','-20.44','-20.44','20.48';'Internal_used','14','8','LE','unsigned','Multiplexed','0','1','0','-Inf','Inf';'Internal_used2','32','7','LE','unsigned','Multiplexed','0','1','0','-Inf','Inf';'Internal_used3','51','7','LE','unsigned','Multiplexed','0','1','0','-Inf','Inf';'Internal_used4','58','6','LE','unsigned','Multiplexed','0','1','0','-Inf','Inf';'Internal_used5','9','8','LE','unsigned','Multiplexed','1','1','0','-Inf','Inf';'Internal_used6','17','8','LE','unsigned','Multiplexed','1','1','0','-Inf','Inf';'Internal_used7','25','7','LE','unsigned','Multiplexed','1','1','0','-Inf','Inf';'Mode_Signal','0','1','LE','unsigned','Multiplexor','0','1','0','0','1';'RCS','1','7','LE','unsigned','Multiplexed','1','0.2','-15','-15','36';'Range1','1','13','LE','unsigned','Multiplexed','0','0.04','0','0','327.64';'Reserve_3','32','5','LE','unsigned','Multiplexed','1','1','0','-Inf','Inf';'Reserve_4','47','16','LE','unsigned','Multiplexed','1','1','0','-Inf','Inf';'Speed_Radial','39','12','LE','unsigned','Multiplexed','0','0.04','-119.68','-44.12','119.68'}  IDPort=on  TimestampPort=on  ErrorPort=off  RemotePort=off  LengthPort=off  StatusPort=off  ApplyMinMax=off
      settings: DataFormat=CANdb specified signals
  CAN Unpack119 : canmsglib/CAN Unpack  CANdbFile=eWolf_SensorCAN.dbc  MsgList=Radar_RawTarget_Data_118  MsgName=Radar_RawTarget_Data_118  MsgIDType=Standard (11-bit identifier)  MsgIdentifier=1142  MsgLength=8  SignalInfo={'AZ_Winkel','22','10','LE','unsigned','Multiplexed','0','0.16','-81.76','-81.76','81.92';'EL_Angle','37','10','LE','unsigned','Multiplexed','1','0.04','-20.44','-20.44','20.48';'Internal_used','14','8','LE','unsigned','Multiplexed','0','1','0','-Inf','Inf';'Internal_used2','32','7','LE','unsigned','Multiplexed','0','1','0','-Inf','Inf';'Internal_used3','51','7','LE','unsigned','Multiplexed','0','1','0','-Inf','Inf';'Internal_used4','58','6','LE','unsigned','Multiplexed','0','1','0','-Inf','Inf';'Internal_used5','9','8','LE','unsigned','Multiplexed','1','1','0','-Inf','Inf';'Internal_used6','17','8','LE','unsigned','Multiplexed','1','1','0','-Inf','Inf';'Internal_used7','25','7','LE','unsigned','Multiplexed','1','1','0','-Inf','Inf';'Mode_Signal','0','1','LE','unsigned','Multiplexor','0','1','0','0','1';'RCS','1','7','LE','unsigned','Multiplexed','1','0.2','-15','-15','36';'Range1','1','13','LE','unsigned','Multiplexed','0','0.04','0','0','327.64';'Reserve_3','32','5','LE','unsigned','Multiplexed','1','1','0','-Inf','Inf';'Reserve_4','47','16','LE','unsigned','Multiplexed','1','1','0','-Inf','Inf';'Speed_Radial','39','12','LE','unsigned','Multiplexed','0','0.04','-119.68','-44.12','119.68'}  IDPort=on  TimestampPort=on  ErrorPort=off  RemotePort=off  LengthPort=off  StatusPort=off  ApplyMinMax=off
      settings: DataFormat=CANdb specified signals
  CAN Unpack12 : canmsglib/CAN Unpack  CANdbFile=eWolf_SensorCAN.dbc  MsgList=Radar_RawTarget_Data_011  MsgName=Radar_RawTarget_Data_011  MsgIDType=Standard (11-bit identifier)  MsgIdentifier=1035  MsgLength=8  SignalInfo={'AZ_Winkel','22','10','LE','unsigned','Multiplexed','0','0.16','-81.76','-81.76','81.92';'EL_Angle','37','10','LE','unsigned','Multiplexed','1','0.04','-20.44','-20.44','20.48';'Internal_used','14','8','LE','unsigned','Multiplexed','0','1','0','-Inf','Inf';'Internal_used2','32','7','LE','unsigned','Multiplexed','0','1','0','-Inf','Inf';'Internal_used3','51','7','LE','unsigned','Multiplexed','0','1','0','-Inf','Inf';'Internal_used4','58','6','LE','unsigned','Multiplexed','0','1','0','-Inf','Inf';'Internal_used5','9','8','LE','unsigned','Multiplexed','1','1','0','-Inf','Inf';'Internal_used6','17','8','LE','unsigned','Multiplexed','1','1','0','-Inf','Inf';'Internal_used7','25','7','LE','unsigned','Multiplexed','1','1','0','-Inf','Inf';'Mode_Signal','0','1','LE','unsigned','Multiplexor','0','1','0','0','1';'RCS','1','7','LE','unsigned','Multiplexed','1','0.2','-15','-15','36';'Range1','1','13','LE','unsigned','Multiplexed','0','0.04','0','0','327.64';'Reserve_3','32','5','LE','unsigned','Multiplexed','1','1','0','-Inf','Inf';'Reserve_4','47','16','LE','unsigned','Multiplexed','1','1','0','-Inf','Inf';'Speed_Radial','39','12','LE','unsigned','Multiplexed','0','0.04','-119.68','-44.12','119.68'}  IDPort=on  TimestampPort=on  ErrorPort=off  RemotePort=off  LengthPort=off  StatusPort=off  ApplyMinMax=off
      settings: DataFormat=CANdb specified signals
  CAN Unpack120 : canmsglib/CAN Unpack  CANdbFile=eWolf_SensorCAN.dbc  MsgList=Radar_RawTarget_Data_119  MsgName=Radar_RawTarget_Data_119  MsgIDType=Standard (11-bit identifier)  MsgIdentifier=1143  MsgLength=8  SignalInfo={'AZ_Winkel','22','10','LE','unsigned','Multiplexed','0','0.16','-81.76','-81.76','81.92';'EL_Angle','37','10','LE','unsigned','Multiplexed','1','0.04','-20.44','-20.44','20.48';'Internal_used','14','8','LE','unsigned','Multiplexed','0','1','0','-Inf','Inf';'Internal_used2','32','7','LE','unsigned','Multiplexed','0','1','0','-Inf','Inf';'Internal_used3','51','7','LE','unsigned','Multiplexed','0','1','0','-Inf','Inf';'Internal_used4','58','6','LE','unsigned','Multiplexed','0','1','0','-Inf','Inf';'Internal_used5','9','8','LE','unsigned','Multiplexed','1','1','0','-Inf','Inf';'Internal_used6','17','8','LE','unsigned','Multiplexed','1','1','0','-Inf','Inf';'Internal_used7','25','7','LE','unsigned','Multiplexed','1','1','0','-Inf','Inf';'Mode_Signal','0','1','LE','unsigned','Multiplexor','0','1','0','0','1';'RCS','1','7','LE','unsigned','Multiplexed','1','0.2','-15','-15','36';'Range1','1','13','LE','unsigned','Multiplexed','0','0.04','0','0','327.64';'Reserve_3','32','5','LE','unsigned','Multiplexed','1','1','0','-Inf','Inf';'Reserve_4','47','16','LE','unsigned','Multiplexed','1','1','0','-Inf','Inf';'Speed_Radial','39','12','LE','unsigned','Multiplexed','0','0.04','-119.68','-44.12','119.68'}  IDPort=on  TimestampPort=on  ErrorPort=off  RemotePort=off  LengthPort=off  StatusPort=off  ApplyMinMax=off
      settings: DataFormat=CANdb specified signals
  CAN Unpack121 : canmsglib/CAN Unpack  CANdbFile=eWolf_SensorCAN.dbc  MsgList=Radar_RawTarget_Data_120  MsgName=Radar_RawTarget_Data_120  MsgIDType=Standard (11-bit identifier)  MsgIdentifier=1144  MsgLength=8  SignalInfo={'AZ_Winkel','22','10','LE','unsigned','Multiplexed','0','0.16','-81.76','-81.76','81.92';'EL_Angle','37','10','LE','unsigned','Multiplexed','1','0.04','-20.44','-20.44','20.48';'Internal_used','14','8','LE','unsigned','Multiplexed','0','1','0','-Inf','Inf';'Internal_used2','32','7','LE','unsigned','Multiplexed','0','1','0','-Inf','Inf';'Internal_used3','51','7','LE','unsigned','Multiplexed','0','1','0','-Inf','Inf';'Internal_used4','58','6','LE','unsigned','Multiplexed','0','1','0','-Inf','Inf';'Internal_used5','9','8','LE','unsigned','Multiplexed','1','1','0','-Inf','Inf';'Internal_used6','17','8','LE','unsigned','Multiplexed','1','1','0','-Inf','Inf';'Internal_used7','25','7','LE','unsigned','Multiplexed','1','1','0','-Inf','Inf';'Mode_Signal','0','1','LE','unsigned','Multiplexor','0','1','0','0','1';'RCS','1','7','LE','unsigned','Multiplexed','1','0.2','-15','-15','36';'Range1','1','13','LE','unsigned','Multiplexed','0','0.04','0','0','327.64';'Reserve_3','32','5','LE','unsigned','Multiplexed','1','1','0','-Inf','Inf';'Reserve_4','47','16','LE','unsigned','Multiplexed','1','1','0','-Inf','Inf';'Speed_Radial','39','12','LE','unsigned','Multiplexed','0','0.04','-119.68','-44.12','119.68'}  IDPort=on  TimestampPort=on  ErrorPort=off  RemotePort=off  LengthPort=off  StatusPort=off  ApplyMinMax=off
      settings: DataFormat=CANdb specified signals
  CAN Unpack122 : canmsglib/CAN Unpack  CANdbFile=eWolf_SensorCAN.dbc  MsgList=Radar_RawTarget_Data_121  MsgName=Radar_RawTarget_Data_121  MsgIDType=Standard (11-bit identifier)  MsgIdentifier=1145  MsgLength=8  SignalInfo={'AZ_Winkel','22','10','LE','unsigned','Multiplexed','0','0.16','-81.76','-81.76','81.92';'EL_Angle','37','10','LE','unsigned','Multiplexed','1','0.04','-20.44','-20.44','20.48';'Internal_used','14','8','LE','unsigned','Multiplexed','0','1','0','-Inf','Inf';'Internal_used2','32','7','LE','unsigned','Multiplexed','0','1','0','-Inf','Inf';'Internal_used3','51','7','LE','unsigned','Multiplexed','0','1','0','-Inf','Inf';'Internal_used4','58','6','LE','unsigned','Multiplexed','0','1','0','-Inf','Inf';'Internal_used5','9','8','LE','unsigned','Multiplexed','1','1','0','-Inf','Inf';'Internal_used6','17','8','LE','unsigned','Multiplexed','1','1','0','-Inf','Inf';'Internal_used7','25','7','LE','unsigned','Multiplexed','1','1','0','-Inf','Inf';'Mode_Signal','0','1','LE','unsigned','Multiplexor','0','1','0','0','1';'RCS','1','7','LE','unsigned','Multiplexed','1','0.2','-15','-15','36';'Range1','1','13','LE','unsigned','Multiplexed','0','0.04','0','0','327.64';'Reserve_3','32','5','LE','unsigned','Multiplexed','1','1','0','-Inf','Inf';'Reserve_4','47','16','LE','unsigned','Multiplexed','1','1','0','-Inf','Inf';'Speed_Radial','39','12','LE','unsigned','Multiplexed','0','0.04','-119.68','-44.12','119.68'}  IDPort=on  TimestampPort=on  ErrorPort=off  RemotePort=off  LengthPort=off  StatusPort=off  ApplyMinMax=off
      settings: DataFormat=CANdb specified signals
  CAN Unpack123 : canmsglib/CAN Unpack  CANdbFile=eWolf_SensorCAN.dbc  MsgList=Radar_RawTarget_Data_122  MsgName=Radar_RawTarget_Data_122  MsgIDType=Standard (11-bit identifier)  MsgIdentifier=1146  MsgLength=8  SignalInfo={'AZ_Winkel','22','10','LE','unsigned','Multiplexed','0','0.16','-81.76','-81.76','81.92';'EL_Angle','37','10','LE','unsigned','Multiplexed','1','0.04','-20.44','-20.44','20.48';'Internal_used','14','8','LE','unsigned','Multiplexed','0','1','0','-Inf','Inf';'Internal_used2','32','7','LE','unsigned','Multiplexed','0','1','0','-Inf','Inf';'Internal_used3','51','7','LE','unsigned','Multiplexed','0','1','0','-Inf','Inf';'Internal_used4','58','6','LE','unsigned','Multiplexed','0','1','0','-Inf','Inf';'Internal_used5','9','8','LE','unsigned','Multiplexed','1','1','0','-Inf','Inf';'Internal_used6','17','8','LE','unsigned','Multiplexed','1','1','0','-Inf','Inf';'Internal_used7','25','7','LE','unsigned','Multiplexed','1','1','0','-Inf','Inf';'Mode_Signal','0','1','LE','unsigned','Multiplexor','0','1','0','0','1';'RCS','1','7','LE','unsigned','Multiplexed','1','0.2','-15','-15','36';'Range1','1','13','LE','unsigned','Multiplexed','0','0.04','0','0','327.64';'Reserve_3','32','5','LE','unsigned','Multiplexed','1','1','0','-Inf','Inf';'Reserve_4','47','16','LE','unsigned','Multiplexed','1','1','0','-Inf','Inf';'Speed_Radial','39','12','LE','unsigned','Multiplexed','0','0.04','-119.68','-44.12','119.68'}  IDPort=on  TimestampPort=on  ErrorPort=off  RemotePort=off  LengthPort=off  StatusPort=off  ApplyMinMax=off
      settings: DataFormat=CANdb specified signals
  CAN Unpack124 : canmsglib/CAN Unpack  CANdbFile=eWolf_SensorCAN.dbc  MsgList=Radar_RawTarget_Data_123  MsgName=Radar_RawTarget_Data_123  MsgIDType=Standard (11-bit identifier)  MsgIdentifier=1147  MsgLength=8  SignalInfo={'AZ_Winkel','22','10','LE','unsigned','Multiplexed','0','0.16','-81.76','-81.76','81.92';'EL_Angle','37','10','LE','unsigned','Multiplexed','1','0.04','-20.44','-20.44','20.48';'Internal_used','14','8','LE','unsigned','Multiplexed','0','1','0','-Inf','Inf';'Internal_used2','32','7','LE','unsigned','Multiplexed','0','1','0','-Inf','Inf';'Internal_used3','51','7','LE','unsigned','Multiplexed','0','1','0','-Inf','Inf';'Internal_used4','58','6','LE','unsigned','Multiplexed','0','1','0','-Inf','Inf';'Internal_used5','9','8','LE','unsigned','Multiplexed','1','1','0','-Inf','Inf';'Internal_used6','17','8','LE','unsigned','Multiplexed','1','1','0','-Inf','Inf';'Internal_used7','25','7','LE','unsigned','Multiplexed','1','1','0','-Inf','Inf';'Mode_Signal','0','1','LE','unsigned','Multiplexor','0','1','0','0','1';'RCS','1','7','LE','unsigned','Multiplexed','1','0.2','-15','-15','36';'Range1','1','13','LE','unsigned','Multiplexed','0','0.04','0','0','327.64';'Reserve_3','32','5','LE','unsigned','Multiplexed','1','1','0','-Inf','Inf';'Reserve_4','47','16','LE','unsigned','Multiplexed','1','1','0','-Inf','Inf';'Speed_Radial','39','12','LE','unsigned','Multiplexed','0','0.04','-119.68','-44.12','119.68'}  IDPort=on  TimestampPort=on  ErrorPort=off  RemotePort=off  LengthPort=off  StatusPort=off  ApplyMinMax=off
      settings: DataFormat=CANdb specified signals
  CAN Unpack125 : canmsglib/CAN Unpack  CANdbFile=eWolf_SensorCAN.dbc  MsgList=Radar_RawTarget_Data_124  MsgName=Radar_RawTarget_Data_124  MsgIDType=Standard (11-bit identifier)  MsgIdentifier=1148  MsgLength=8  SignalInfo={'AZ_Winkel','22','10','LE','unsigned','Multiplexed','0','0.16','-81.76','-81.76','81.92';'EL_Angle','37','10','LE','unsigned','Multiplexed','1','0.04','-20.44','-20.44','20.48';'Internal_used','14','8','LE','unsigned','Multiplexed','0','1','0','-Inf','Inf';'Internal_used2','32','7','LE','unsigned','Multiplexed','0','1','0','-Inf','Inf';'Internal_used3','51','7','LE','unsigned','Multiplexed','0','1','0','-Inf','Inf';'Internal_used4','58','6','LE','unsigned','Multiplexed','0','1','0','-Inf','Inf';'Internal_used5','9','8','LE','unsigned','Multiplexed','1','1','0','-Inf','Inf';'Internal_used6','17','8','LE','unsigned','Multiplexed','1','1','0','-Inf','Inf';'Internal_used7','25','7','LE','unsigned','Multiplexed','1','1','0','-Inf','Inf';'Mode_Signal','0','1','LE','unsigned','Multiplexor','0','1','0','0','1';'RCS','1','7','LE','unsigned','Multiplexed','1','0.2','-15','-15','36';'Range1','1','13','LE','unsigned','Multiplexed','0','0.04','0','0','327.64';'Reserve_3','32','5','LE','unsigned','Multiplexed','1','1','0','-Inf','Inf';'Reserve_4','47','16','LE','unsigned','Multiplexed','1','1','0','-Inf','Inf';'Speed_Radial','39','12','LE','unsigned','Multiplexed','0','0.04','-119.68','-44.12','119.68'}  IDPort=on  TimestampPort=on  ErrorPort=off  RemotePort=off  LengthPort=off  StatusPort=off  ApplyMinMax=off
      settings: DataFormat=CANdb specified signals
  CAN Unpack126 : canmsglib/CAN Unpack  CANdbFile=eWolf_SensorCAN.dbc  MsgList=Radar_RawTarget_Data_125  MsgName=Radar_RawTarget_Data_125  MsgIDType=Standard (11-bit identifier)  MsgIdentifier=1149  MsgLength=8  SignalInfo={'AZ_Winkel','22','10','LE','unsigned','Multiplexed','0','0.16','-81.76','-81.76','81.92';'EL_Angle','37','10','LE','unsigned','Multiplexed','1','0.04','-20.44','-20.44','20.48';'Internal_used','14','8','LE','unsigned','Multiplexed','0','1','0','-Inf','Inf';'Internal_used2','32','7','LE','unsigned','Multiplexed','0','1','0','-Inf','Inf';'Internal_used3','51','7','LE','unsigned','Multiplexed','0','1','0','-Inf','Inf';'Internal_used4','58','6','LE','unsigned','Multiplexed','0','1','0','-Inf','Inf';'Internal_used5','9','8','LE','unsigned','Multiplexed','1','1','0','-Inf','Inf';'Internal_used6','17','8','LE','unsigned','Multiplexed','1','1','0','-Inf','Inf';'Internal_used7','25','7','LE','unsigned','Multiplexed','1','1','0','-Inf','Inf';'Mode_Signal','0','1','LE','unsigned','Multiplexor','0','1','0','0','1';'RCS','1','7','LE','unsigned','Multiplexed','1','0.2','-15','-15','36';'Range1','1','13','LE','unsigned','Multiplexed','0','0.04','0','0','327.64';'Reserve_3','32','5','LE','unsigned','Multiplexed','1','1','0','-Inf','Inf';'Reserve_4','47','16','LE','unsigned','Multiplexed','1','1','0','-Inf','Inf';'Speed_Radial','39','12','LE','unsigned','Multiplexed','0','0.04','-119.68','-44.12','119.68'}  IDPort=on  TimestampPort=on  ErrorPort=off  RemotePort=off  LengthPort=off  StatusPort=off  ApplyMinMax=off
      settings: DataFormat=CANdb specified signals
  CAN Unpack127 : canmsglib/CAN Unpack  CANdbFile=eWolf_SensorCAN.dbc  MsgList=Radar_RawTarget_Data_126  MsgName=Radar_RawTarget_Data_126  MsgIDType=Standard (11-bit identifier)  MsgIdentifier=1150  MsgLength=8  SignalInfo={'AZ_Winkel','22','10','LE','unsigned','Multiplexed','0','0.16','-81.76','-81.76','81.92';'EL_Angle','37','10','LE','unsigned','Multiplexed','1','0.04','-20.44','-20.44','20.48';'Internal_used','14','8','LE','unsigned','Multiplexed','0','1','0','-Inf','Inf';'Internal_used2','32','7','LE','unsigned','Multiplexed','0','1','0','-Inf','Inf';'Internal_used3','51','7','LE','unsigned','Multiplexed','0','1','0','-Inf','Inf';'Internal_used4','58','6','LE','unsigned','Multiplexed','0','1','0','-Inf','Inf';'Internal_used5','9','8','LE','unsigned','Multiplexed','1','1','0','-Inf','Inf';'Internal_used6','17','8','LE','unsigned','Multiplexed','1','1','0','-Inf','Inf';'Internal_used7','25','7','LE','unsigned','Multiplexed','1','1','0','-Inf','Inf';'Mode_Signal','0','1','LE','unsigned','Multiplexor','0','1','0','0','1';'RCS','1','7','LE','unsigned','Multiplexed','1','0.2','-15','-15','36';'Range1','1','13','LE','unsigned','Multiplexed','0','0.04','0','0','327.64';'Reserve_3','32','5','LE','unsigned','Multiplexed','1','1','0','-Inf','Inf';'Reserve_4','47','16','LE','unsigned','Multiplexed','1','1','0','-Inf','Inf';'Speed_Radial','39','12','LE','unsigned','Multiplexed','0','0.04','-119.68','-44.12','119.68'}  IDPort=on  TimestampPort=on  ErrorPort=off  RemotePort=off  LengthPort=off  StatusPort=off  ApplyMinMax=off
      settings: DataFormat=CANdb specified signals
  CAN Unpack128 : canmsglib/CAN Unpack  CANdbFile=eWolf_SensorCAN.dbc  MsgList=Radar_RawTarget_Data_127  MsgName=Radar_RawTarget_Data_127  MsgIDType=Standard (11-bit identifier)  MsgIdentifier=1151  MsgLength=8  SignalInfo={'AZ_Winkel','22','10','LE','unsigned','Multiplexed','0','0.16','-81.76','-81.76','81.92';'EL_Angle','37','10','LE','unsigned','Multiplexed','1','0.04','-20.44','-20.44','20.48';'Internal_used','14','8','LE','unsigned','Multiplexed','0','1','0','-Inf','Inf';'Internal_used2','32','7','LE','unsigned','Multiplexed','0','1','0','-Inf','Inf';'Internal_used3','51','7','LE','unsigned','Multiplexed','0','1','0','-Inf','Inf';'Internal_used4','58','6','LE','unsigned','Multiplexed','0','1','0','-Inf','Inf';'Internal_used5','9','8','LE','unsigned','Multiplexed','1','1','0','-Inf','Inf';'Internal_used6','17','8','LE','unsigned','Multiplexed','1','1','0','-Inf','Inf';'Internal_used7','25','7','LE','unsigned','Multiplexed','1','1','0','-Inf','Inf';'Mode_Signal','0','1','LE','unsigned','Multiplexor','0','1','0','0','1';'RCS','1','7','LE','unsigned','Multiplexed','1','0.2','-15','-15','36';'Range1','1','13','LE','unsigned','Multiplexed','0','0.04','0','0','327.64';'Reserve_3','32','5','LE','unsigned','Multiplexed','1','1','0','-Inf','Inf';'Reserve_4','47','16','LE','unsigned','Multiplexed','1','1','0','-Inf','Inf';'Speed_Radial','39','12','LE','unsigned','Multiplexed','0','0.04','-119.68','-44.12','119.68'}  IDPort=on  TimestampPort=on  ErrorPort=off  RemotePort=off  LengthPort=off  StatusPort=off  ApplyMinMax=off
      settings: DataFormat=CANdb specified signals
  CAN Unpack129 : canmsglib/CAN Unpack  CANdbFile=eWolf_SensorCAN.dbc  MsgList=Radar_RawTarget_Data_128  MsgName=Radar_RawTarget_Data_128  MsgIDType=Standard (11-bit identifier)  MsgIdentifier=1152  MsgLength=8  SignalInfo={'AZ_Winkel','22','10','LE','unsigned','Multiplexed','0','0.16','-81.76','-81.76','81.92';'EL_Angle','37','10','LE','unsigned','Multiplexed','1','0.04','-20.44','-20.44','20.48';'Internal_used','14','8','LE','unsigned','Multiplexed','0','1','0','-Inf','Inf';'Internal_used2','32','7','LE','unsigned','Multiplexed','0','1','0','-Inf','Inf';'Internal_used3','51','7','LE','unsigned','Multiplexed','0','1','0','-Inf','Inf';'Internal_used4','58','6','LE','unsigned','Multiplexed','0','1','0','-Inf','Inf';'Internal_used5','9','8','LE','unsigned','Multiplexed','1','1','0','-Inf','Inf';'Internal_used6','17','8','LE','unsigned','Multiplexed','1','1','0','-Inf','Inf';'Internal_used7','25','7','LE','unsigned','Multiplexed','1','1','0','-Inf','Inf';'Mode_Signal','0','1','LE','unsigned','Multiplexor','0','1','0','0','1';'RCS','1','7','LE','unsigned','Multiplexed','1','0.2','-15','-15','36';'Range1','1','13','LE','unsigned','Multiplexed','0','0.04','0','0','327.64';'Reserve_3','32','5','LE','unsigned','Multiplexed','1','1','0','-Inf','Inf';'Reserve_4','47','16','LE','unsigned','Multiplexed','1','1','0','-Inf','Inf';'Speed_Radial','39','12','LE','unsigned','Multiplexed','0','0.04','-119.68','-44.12','119.68'}  IDPort=on  TimestampPort=on  ErrorPort=off  RemotePort=off  LengthPort=off  StatusPort=off  ApplyMinMax=off
      settings: DataFormat=CANdb specified signals
  CAN Unpack13 : canmsglib/CAN Unpack  CANdbFile=eWolf_SensorCAN.dbc  MsgList=Radar_RawTarget_Data_012  MsgName=Radar_RawTarget_Data_012  MsgIDType=Standard (11-bit identifier)  MsgIdentifier=1036  MsgLength=8  SignalInfo={'AZ_Winkel','22','10','LE','unsigned','Multiplexed','0','0.16','-81.76','-81.76','81.92';'EL_Angle','37','10','LE','unsigned','Multiplexed','1','0.04','-20.44','-20.44','20.48';'Internal_used','14','8','LE','unsigned','Multiplexed','0','1','0','-Inf','Inf';'Internal_used2','32','7','LE','unsigned','Multiplexed','0','1','0','-Inf','Inf';'Internal_used3','51','7','LE','unsigned','Multiplexed','0','1','0','-Inf','Inf';'Internal_used4','58','6','LE','unsigned','Multiplexed','0','1','0','-Inf','Inf';'Internal_used5','9','8','LE','unsigned','Multiplexed','1','1','0','-Inf','Inf';'Internal_used6','17','8','LE','unsigned','Multiplexed','1','1','0','-Inf','Inf';'Internal_used7','25','7','LE','unsigned','Multiplexed','1','1','0','-Inf','Inf';'Mode_Signal','0','1','LE','unsigned','Multiplexor','0','1','0','0','1';'RCS','1','7','LE','unsigned','Multiplexed','1','0.2','-15','-15','36';'Range1','1','13','LE','unsigned','Multiplexed','0','0.04','0','0','327.64';'Reserve_3','32','5','LE','unsigned','Multiplexed','1','1','0','-Inf','Inf';'Reserve_4','47','16','LE','unsigned','Multiplexed','1','1','0','-Inf','Inf';'Speed_Radial','39','12','LE','unsigned','Multiplexed','0','0.04','-119.68','-44.12','119.68'}  IDPort=on  TimestampPort=on  ErrorPort=off  RemotePort=off  LengthPort=off  StatusPort=off  ApplyMinMax=off
      settings: DataFormat=CANdb specified signals
  CAN Unpack14 : canmsglib/CAN Unpack  CANdbFile=eWolf_SensorCAN.dbc  MsgList=Radar_RawTarget_Data_013  MsgName=Radar_RawTarget_Data_013  MsgIDType=Standard (11-bit identifier)  MsgIdentifier=1037  MsgLength=8  SignalInfo={'AZ_Winkel','22','10','LE','unsigned','Multiplexed','0','0.16','-81.76','-81.76','81.92';'EL_Angle','37','10','LE','unsigned','Multiplexed','1','0.04','-20.44','-20.44','20.48';'Internal_used','14','8','LE','unsigned','Multiplexed','0','1','0','-Inf','Inf';'Internal_used2','32','7','LE','unsigned','Multiplexed','0','1','0','-Inf','Inf';'Internal_used3','51','7','LE','unsigned','Multiplexed','0','1','0','-Inf','Inf';'Internal_used4','58','6','LE','unsigned','Multiplexed','0','1','0','-Inf','Inf';'Internal_used5','9','8','LE','unsigned','Multiplexed','1','1','0','-Inf','Inf';'Internal_used6','17','8','LE','unsigned','Multiplexed','1','1','0','-Inf','Inf';'Internal_used7','25','7','LE','unsigned','Multiplexed','1','1','0','-Inf','Inf';'Mode_Signal','0','1','LE','unsigned','Multiplexor','0','1','0','0','1';'RCS','1','7','LE','unsigned','Multiplexed','1','0.2','-15','-15','36';'Range1','1','13','LE','unsigned','Multiplexed','0','0.04','0','0','327.64';'Reserve_3','32','5','LE','unsigned','Multiplexed','1','1','0','-Inf','Inf';'Reserve_4','47','16','LE','unsigned','Multiplexed','1','1','0','-Inf','Inf';'Speed_Radial','39','12','LE','unsigned','Multiplexed','0','0.04','-119.68','-44.12','119.68'}  IDPort=on  TimestampPort=on  ErrorPort=off  RemotePort=off  LengthPort=off  StatusPort=off  ApplyMinMax=off
      settings: DataFormat=CANdb specified signals
  CAN Unpack15 : canmsglib/CAN Unpack  CANdbFile=eWolf_SensorCAN.dbc  MsgList=Radar_RawTarget_Data_014  MsgName=Radar_RawTarget_Data_014  MsgIDType=Standard (11-bit identifier)  MsgIdentifier=1038  MsgLength=8  SignalInfo={'AZ_Winkel','22','10','LE','unsigned','Multiplexed','0','0.16','-81.76','-81.76','81.92';'EL_Angle','37','10','LE','unsigned','Multiplexed','1','0.04','-20.44','-20.44','20.48';'Internal_used','14','8','LE','unsigned','Multiplexed','0','1','0','-Inf','Inf';'Internal_used2','32','7','LE','unsigned','Multiplexed','0','1','0','-Inf','Inf';'Internal_used3','51','7','LE','unsigned','Multiplexed','0','1','0','-Inf','Inf';'Internal_used4','58','6','LE','unsigned','Multiplexed','0','1','0','-Inf','Inf';'Internal_used5','9','8','LE','unsigned','Multiplexed','1','1','0','-Inf','Inf';'Internal_used6','17','8','LE','unsigned','Multiplexed','1','1','0','-Inf','Inf';'Internal_used7','25','7','LE','unsigned','Multiplexed','1','1','0','-Inf','Inf';'Mode_Signal','0','1','LE','unsigned','Multiplexor','0','1','0','0','1';'RCS','1','7','LE','unsigned','Multiplexed','1','0.2','-15','-15','36';'Range1','1','13','LE','unsigned','Multiplexed','0','0.04','0','0','327.64';'Reserve_3','32','5','LE','unsigned','Multiplexed','1','1','0','-Inf','Inf';'Reserve_4','47','16','LE','unsigned','Multiplexed','1','1','0','-Inf','Inf';'Speed_Radial','39','12','LE','unsigned','Multiplexed','0','0.04','-119.68','-44.12','119.68'}  IDPort=on  TimestampPort=on  ErrorPort=off  RemotePort=off  LengthPort=off  StatusPort=off  ApplyMinMax=off
      settings: DataFormat=CANdb specified signals
  CAN Unpack16 : canmsglib/CAN Unpack  CANdbFile=eWolf_SensorCAN.dbc  MsgList=Radar_RawTarget_Data_015  MsgName=Radar_RawTarget_Data_015  MsgIDType=Standard (11-bit identifier)  MsgIdentifier=1039  MsgLength=8  SignalInfo={'AZ_Winkel','22','10','LE','unsigned','Multiplexed','0','0.16','-81.76','-81.76','81.92';'EL_Angle','37','10','LE','unsigned','Multiplexed','1','0.04','-20.44','-20.44','20.48';'Internal_used','14','8','LE','unsigned','Multiplexed','0','1','0','-Inf','Inf';'Internal_used2','32','7','LE','unsigned','Multiplexed','0','1','0','-Inf','Inf';'Internal_used3','51','7','LE','unsigned','Multiplexed','0','1','0','-Inf','Inf';'Internal_used4','58','6','LE','unsigned','Multiplexed','0','1','0','-Inf','Inf';'Internal_used5','9','8','LE','unsigned','Multiplexed','1','1','0','-Inf','Inf';'Internal_used6','17','8','LE','unsigned','Multiplexed','1','1','0','-Inf','Inf';'Internal_used7','25','7','LE','unsigned','Multiplexed','1','1','0','-Inf','Inf';'Mode_Signal','0','1','LE','unsigned','Multiplexor','0','1','0','0','1';'RCS','1','7','LE','unsigned','Multiplexed','1','0.2','-15','-15','36';'Range1','1','13','LE','unsigned','Multiplexed','0','0.04','0','0','327.64';'Reserve_3','32','5','LE','unsigned','Multiplexed','1','1','0','-Inf','Inf';'Reserve_4','47','16','LE','unsigned','Multiplexed','1','1','0','-Inf','Inf';'Speed_Radial','39','12','LE','unsigned','Multiplexed','0','0.04','-119.68','-44.12','119.68'}  IDPort=on  TimestampPort=on  ErrorPort=off  RemotePort=off  LengthPort=off  StatusPort=off  ApplyMinMax=off
      settings: DataFormat=CANdb specified signals
  CAN Unpack17 : canmsglib/CAN Unpack  CANdbFile=eWolf_SensorCAN.dbc  MsgList=Radar_RawTarget_Data_016  MsgName=Radar_RawTarget_Data_016  MsgIDType=Standard (11-bit identifier)  MsgIdentifier=1040  MsgLength=8  SignalInfo={'AZ_Winkel','22','10','LE','unsigned','Multiplexed','0','0.16','-81.76','-81.76','81.92';'EL_Angle','37','10','LE','unsigned','Multiplexed','1','0.04','-20.44','-20.44','20.48';'Internal_used','14','8','LE','unsigned','Multiplexed','0','1','0','-Inf','Inf';'Internal_used2','32','7','LE','unsigned','Multiplexed','0','1','0','-Inf','Inf';'Internal_used3','51','7','LE','unsigned','Multiplexed','0','1','0','-Inf','Inf';'Internal_used4','58','6','LE','unsigned','Multiplexed','0','1','0','-Inf','Inf';'Internal_used5','9','8','LE','unsigned','Multiplexed','1','1','0','-Inf','Inf';'Internal_used6','17','8','LE','unsigned','Multiplexed','1','1','0','-Inf','Inf';'Internal_used7','25','7','LE','unsigned','Multiplexed','1','1','0','-Inf','Inf';'Mode_Signal','0','1','LE','unsigned','Multiplexor','0','1','0','0','1';'RCS','1','7','LE','unsigned','Multiplexed','1','0.2','-15','-15','36';'Range1','1','13','LE','unsigned','Multiplexed','0','0.04','0','0','327.64';'Reserve_3','32','5','LE','unsigned','Multiplexed','1','1','0','-Inf','Inf';'Reserve_4','47','16','LE','unsigned','Multiplexed','1','1','0','-Inf','Inf';'Speed_Radial','39','12','LE','unsigned','Multiplexed','0','0.04','-119.68','-44.12','119.68'}  IDPort=on  TimestampPort=on  ErrorPort=off  RemotePort=off  LengthPort=off  StatusPort=off  ApplyMinMax=off
      settings: DataFormat=CANdb specified signals
  CAN Unpack18 : canmsglib/CAN Unpack  CANdbFile=eWolf_SensorCAN.dbc  MsgList=Radar_RawTarget_Data_017  MsgName=Radar_RawTarget_Data_017  MsgIDType=Standard (11-bit identifier)  MsgIdentifier=1041  MsgLength=8  SignalInfo={'AZ_Winkel','22','10','LE','unsigned','Multiplexed','0','0.16','-81.76','-81.76','81.92';'EL_Angle','37','10','LE','unsigned','Multiplexed','1','0.04','-20.44','-20.44','20.48';'Internal_used','14','8','LE','unsigned','Multiplexed','0','1','0','-Inf','Inf';'Internal_used2','32','7','LE','unsigned','Multiplexed','0','1','0','-Inf','Inf';'Internal_used3','51','7','LE','unsigned','Multiplexed','0','1','0','-Inf','Inf';'Internal_used4','58','6','LE','unsigned','Multiplexed','0','1','0','-Inf','Inf';'Internal_used5','9','8','LE','unsigned','Multiplexed','1','1','0','-Inf','Inf';'Internal_used6','17','8','LE','unsigned','Multiplexed','1','1','0','-Inf','Inf';'Internal_used7','25','7','LE','unsigned','Multiplexed','1','1','0','-Inf','Inf';'Mode_Signal','0','1','LE','unsigned','Multiplexor','0','1','0','0','1';'RCS','1','7','LE','unsigned','Multiplexed','1','0.2','-15','-15','36';'Range1','1','13','LE','unsigned','Multiplexed','0','0.04','0','0','327.64';'Reserve_3','32','5','LE','unsigned','Multiplexed','1','1','0','-Inf','Inf';'Reserve_4','47','16','LE','unsigned','Multiplexed','1','1','0','-Inf','Inf';'Speed_Radial','39','12','LE','unsigned','Multiplexed','0','0.04','-119.68','-44.12','119.68'}  IDPort=on  TimestampPort=on  ErrorPort=off  RemotePort=off  LengthPort=off  StatusPort=off  ApplyMinMax=off
      settings: DataFormat=CANdb specified signals
  CAN Unpack19 : canmsglib/CAN Unpack  CANdbFile=eWolf_SensorCAN.dbc  MsgList=Radar_RawTarget_Data_018  MsgName=Radar_RawTarget_Data_018  MsgIDType=Standard (11-bit identifier)  MsgIdentifier=1042  MsgLength=8  SignalInfo={'AZ_Winkel','22','10','LE','unsigned','Multiplexed','0','0.16','-81.76','-81.76','81.92';'EL_Angle','37','10','LE','unsigned','Multiplexed','1','0.04','-20.44','-20.44','20.48';'Internal_used','14','8','LE','unsigned','Multiplexed','0','1','0','-Inf','Inf';'Internal_used2','32','7','LE','unsigned','Multiplexed','0','1','0','-Inf','Inf';'Internal_used3','51','7','LE','unsigned','Multiplexed','0','1','0','-Inf','Inf';'Internal_used4','58','6','LE','unsigned','Multiplexed','0','1','0','-Inf','Inf';'Internal_used5','9','8','LE','unsigned','Multiplexed','1','1','0','-Inf','Inf';'Internal_used6','17','8','LE','unsigned','Multiplexed','1','1','0','-Inf','Inf';'Internal_used7','25','7','LE','unsigned','Multiplexed','1','1','0','-Inf','Inf';'Mode_Signal','0','1','LE','unsigned','Multiplexor','0','1','0','0','1';'RCS','1','7','LE','unsigned','Multiplexed','1','0.2','-15','-15','36';'Range1','1','13','LE','unsigned','Multiplexed','0','0.04','0','0','327.64';'Reserve_3','32','5','LE','unsigned','Multiplexed','1','1','0','-Inf','Inf';'Reserve_4','47','16','LE','unsigned','Multiplexed','1','1','0','-Inf','Inf';'Speed_Radial','39','12','LE','unsigned','Multiplexed','0','0.04','-119.68','-44.12','119.68'}  IDPort=on  TimestampPort=on  ErrorPort=off  RemotePort=off  LengthPort=off  StatusPort=off  ApplyMinMax=off
      settings: DataFormat=CANdb specified signals
  CAN Unpack2 : canmsglib/CAN Unpack  CANdbFile=eWolf_SensorCAN.dbc  MsgList=Radar_RawTarget_Data_002  MsgName=Radar_RawTarget_Data_002  MsgIDType=Standard (11-bit identifier)  MsgIdentifier=1026  MsgLength=8  SignalInfo={'AZ_Winkel','22','10','LE','unsigned','Multiplexed','0','0.16','-81.76','-81.76','81.92';'EL_Angle','37','10','LE','unsigned','Multiplexed','1','0.04','-20.44','-20.44','20.48';'Internal_used','14','8','LE','unsigned','Multiplexed','0','1','0','-Inf','Inf';'Internal_used2','32','7','LE','unsigned','Multiplexed','0','1','0','-Inf','Inf';'Internal_used3','51','7','LE','unsigned','Multiplexed','0','1','0','-Inf','Inf';'Internal_used4','58','6','LE','unsigned','Multiplexed','0','1','0','-Inf','Inf';'Internal_used5','9','8','LE','unsigned','Multiplexed','1','1','0','-Inf','Inf';'Internal_used6','17','8','LE','unsigned','Multiplexed','1','1','0','-Inf','Inf';'Internal_used7','25','7','LE','unsigned','Multiplexed','1','1','0','-Inf','Inf';'Mode_Signal','0','1','LE','unsigned','Multiplexor','0','1','0','0','1';'RCS','1','7','LE','unsigned','Multiplexed','1','0.2','-15','-15','36';'Range1','1','13','LE','unsigned','Multiplexed','0','0.04','0','0','327.64';'Reserve_3','32','5','LE','unsigned','Multiplexed','1','1','0','-Inf','Inf';'Reserve_4','47','16','LE','unsigned','Multiplexed','1','1','0','-Inf','Inf';'Speed_Radial','39','12','LE','unsigned','Multiplexed','0','0.04','-119.68','-44.12','119.68'}  IDPort=on  TimestampPort=on  ErrorPort=off  RemotePort=off  LengthPort=off  StatusPort=off  ApplyMinMax=off
      settings: DataFormat=CANdb specified signals
  CAN Unpack20 : canmsglib/CAN Unpack  CANdbFile=eWolf_SensorCAN.dbc  MsgList=Radar_RawTarget_Data_019  MsgName=Radar_RawTarget_Data_019  MsgIDType=Standard (11-bit identifier)  MsgIdentifier=1043  MsgLength=8  SignalInfo={'AZ_Winkel','22','10','LE','unsigned','Multiplexed','0','0.16','-81.76','-81.76','81.92';'EL_Angle','37','10','LE','unsigned','Multiplexed','1','0.04','-20.44','-20.44','20.48';'Internal_used','14','8','LE','unsigned','Multiplexed','0','1','0','-Inf','Inf';'Internal_used2','32','7','LE','unsigned','Multiplexed','0','1','0','-Inf','Inf';'Internal_used3','51','7','LE','unsigned','Multiplexed','0','1','0','-Inf','Inf';'Internal_used4','58','6','LE','unsigned','Multiplexed','0','1','0','-Inf','Inf';'Internal_used5','9','8','LE','unsigned','Multiplexed','1','1','0','-Inf','Inf';'Internal_used6','17','8','LE','unsigned','Multiplexed','1','1','0','-Inf','Inf';'Internal_used7','25','7','LE','unsigned','Multiplexed','1','1','0','-Inf','Inf';'Mode_Signal','0','1','LE','unsigned','Multiplexor','0','1','0','0','1';'RCS','1','7','LE','unsigned','Multiplexed','1','0.2','-15','-15','36';'Range1','1','13','LE','unsigned','Multiplexed','0','0.04','0','0','327.64';'Reserve_3','32','5','LE','unsigned','Multiplexed','1','1','0','-Inf','Inf';'Reserve_4','47','16','LE','unsigned','Multiplexed','1','1','0','-Inf','Inf';'Speed_Radial','39','12','LE','unsigned','Multiplexed','0','0.04','-119.68','-44.12','119.68'}  IDPort=on  TimestampPort=on  ErrorPort=off  RemotePort=off  LengthPort=off  StatusPort=off  ApplyMinMax=off
      settings: DataFormat=CANdb specified signals
  CAN Unpack21 : canmsglib/CAN Unpack  CANdbFile=eWolf_SensorCAN.dbc  MsgList=Radar_RawTarget_Data_020  MsgName=Radar_RawTarget_Data_020  MsgIDType=Standard (11-bit identifier)  MsgIdentifier=1044  MsgLength=8  SignalInfo={'AZ_Winkel','22','10','LE','unsigned','Multiplexed','0','0.16','-81.76','-81.76','81.92';'EL_Angle','37','10','LE','unsigned','Multiplexed','1','0.04','-20.44','-20.44','20.48';'Internal_used','14','8','LE','unsigned','Multiplexed','0','1','0','-Inf','Inf';'Internal_used2','32','7','LE','unsigned','Multiplexed','0','1','0','-Inf','Inf';'Internal_used3','51','7','LE','unsigned','Multiplexed','0','1','0','-Inf','Inf';'Internal_used4','58','6','LE','unsigned','Multiplexed','0','1','0','-Inf','Inf';'Internal_used5','9','8','LE','unsigned','Multiplexed','1','1','0','-Inf','Inf';'Internal_used6','17','8','LE','unsigned','Multiplexed','1','1','0','-Inf','Inf';'Internal_used7','25','7','LE','unsigned','Multiplexed','1','1','0','-Inf','Inf';'Mode_Signal','0','1','LE','unsigned','Multiplexor','0','1','0','0','1';'RCS','1','7','LE','unsigned','Multiplexed','1','0.2','-15','-15','36';'Range1','1','13','LE','unsigned','Multiplexed','0','0.04','0','0','327.64';'Reserve_3','32','5','LE','unsigned','Multiplexed','1','1','0','-Inf','Inf';'Reserve_4','47','16','LE','unsigned','Multiplexed','1','1','0','-Inf','Inf';'Speed_Radial','39','12','LE','unsigned','Multiplexed','0','0.04','-119.68','-44.12','119.68'}  IDPort=on  TimestampPort=on  ErrorPort=off  RemotePort=off  LengthPort=off  StatusPort=off  ApplyMinMax=off
      settings: DataFormat=CANdb specified signals
  CAN Unpack22 : canmsglib/CAN Unpack  CANdbFile=eWolf_SensorCAN.dbc  MsgList=Radar_RawTarget_Data_021  MsgName=Radar_RawTarget_Data_021  MsgIDType=Standard (11-bit identifier)  MsgIdentifier=1045  MsgLength=8  SignalInfo={'AZ_Winkel','22','10','LE','unsigned','Multiplexed','0','0.16','-81.76','-81.76','81.92';'EL_Angle','37','10','LE','unsigned','Multiplexed','1','0.04','-20.44','-20.44','20.48';'Internal_used','14','8','LE','unsigned','Multiplexed','0','1','0','-Inf','Inf';'Internal_used2','32','7','LE','unsigned','Multiplexed','0','1','0','-Inf','Inf';'Internal_used3','51','7','LE','unsigned','Multiplexed','0','1','0','-Inf','Inf';'Internal_used4','58','6','LE','unsigned','Multiplexed','0','1','0','-Inf','Inf';'Internal_used5','9','8','LE','unsigned','Multiplexed','1','1','0','-Inf','Inf';'Internal_used6','17','8','LE','unsigned','Multiplexed','1','1','0','-Inf','Inf';'Internal_used7','25','7','LE','unsigned','Multiplexed','1','1','0','-Inf','Inf';'Mode_Signal','0','1','LE','unsigned','Multiplexor','0','1','0','0','1';'RCS','1','7','LE','unsigned','Multiplexed','1','0.2','-15','-15','36';'Range1','1','13','LE','unsigned','Multiplexed','0','0.04','0','0','327.64';'Reserve_3','32','5','LE','unsigned','Multiplexed','1','1','0','-Inf','Inf';'Reserve_4','47','16','LE','unsigned','Multiplexed','1','1','0','-Inf','Inf';'Speed_Radial','39','12','LE','unsigned','Multiplexed','0','0.04','-119.68','-44.12','119.68'}  IDPort=on  TimestampPort=on  ErrorPort=off  RemotePort=off  LengthPort=off  StatusPort=off  ApplyMinMax=off
      settings: DataFormat=CANdb specified signals
  CAN Unpack23 : canmsglib/CAN Unpack  CANdbFile=eWolf_SensorCAN.dbc  MsgList=Radar_RawTarget_Data_022  MsgName=Radar_RawTarget_Data_022  MsgIDType=Standard (11-bit identifier)  MsgIdentifier=1046  MsgLength=8  SignalInfo={'AZ_Winkel','22','10','LE','unsigned','Multiplexed','0','0.16','-81.76','-81.76','81.92';'EL_Angle','37','10','LE','unsigned','Multiplexed','1','0.04','-20.44','-20.44','20.48';'Internal_used','14','8','LE','unsigned','Multiplexed','0','1','0','-Inf','Inf';'Internal_used2','32','7','LE','unsigned','Multiplexed','0','1','0','-Inf','Inf';'Internal_used3','51','7','LE','unsigned','Multiplexed','0','1','0','-Inf','Inf';'Internal_used4','58','6','LE','unsigned','Multiplexed','0','1','0','-Inf','Inf';'Internal_used5','9','8','LE','unsigned','Multiplexed','1','1','0','-Inf','Inf';'Internal_used6','17','8','LE','unsigned','Multiplexed','1','1','0','-Inf','Inf';'Internal_used7','25','7','LE','unsigned','Multiplexed','1','1','0','-Inf','Inf';'Mode_Signal','0','1','LE','unsigned','Multiplexor','0','1','0','0','1';'RCS','1','7','LE','unsigned','Multiplexed','1','0.2','-15','-15','36';'Range1','1','13','LE','unsigned','Multiplexed','0','0.04','0','0','327.64';'Reserve_3','32','5','LE','unsigned','Multiplexed','1','1','0','-Inf','Inf';'Reserve_4','47','16','LE','unsigned','Multiplexed','1','1','0','-Inf','Inf';'Speed_Radial','39','12','LE','unsigned','Multiplexed','0','0.04','-119.68','-44.12','119.68'}  IDPort=on  TimestampPort=on  ErrorPort=off  RemotePort=off  LengthPort=off  StatusPort=off  ApplyMinMax=off
      settings: DataFormat=CANdb specified signals
  CAN Unpack24 : canmsglib/CAN Unpack  CANdbFile=eWolf_SensorCAN.dbc  MsgList=Radar_RawTarget_Data_023  MsgName=Radar_RawTarget_Data_023  MsgIDType=Standard (11-bit identifier)  MsgIdentifier=1047  MsgLength=8  SignalInfo={'AZ_Winkel','22','10','LE','unsigned','Multiplexed','0','0.16','-81.76','-81.76','81.92';'EL_Angle','37','10','LE','unsigned','Multiplexed','1','0.04','-20.44','-20.44','20.48';'Internal_used','14','8','LE','unsigned','Multiplexed','0','1','0','-Inf','Inf';'Internal_used2','32','7','LE','unsigned','Multiplexed','0','1','0','-Inf','Inf';'Internal_used3','51','7','LE','unsigned','Multiplexed','0','1','0','-Inf','Inf';'Internal_used4','58','6','LE','unsigned','Multiplexed','0','1','0','-Inf','Inf';'Internal_used5','9','8','LE','unsigned','Multiplexed','1','1','0','-Inf','Inf';'Internal_used6','17','8','LE','unsigned','Multiplexed','1','1','0','-Inf','Inf';'Internal_used7','25','7','LE','unsigned','Multiplexed','1','1','0','-Inf','Inf';'Mode_Signal','0','1','LE','unsigned','Multiplexor','0','1','0','0','1';'RCS','1','7','LE','unsigned','Multiplexed','1','0.2','-15','-15','36';'Range1','1','13','LE','unsigned','Multiplexed','0','0.04','0','0','327.64';'Reserve_3','32','5','LE','unsigned','Multiplexed','1','1','0','-Inf','Inf';'Reserve_4','47','16','LE','unsigned','Multiplexed','1','1','0','-Inf','Inf';'Speed_Radial','39','12','LE','unsigned','Multiplexed','0','0.04','-119.68','-44.12','119.68'}  IDPort=on  TimestampPort=on  ErrorPort=off  RemotePort=off  LengthPort=off  StatusPort=off  ApplyMinMax=off
      settings: DataFormat=CANdb specified signals
  CAN Unpack25 : canmsglib/CAN Unpack  CANdbFile=eWolf_SensorCAN.dbc  MsgList=Radar_RawTarget_Data_024  MsgName=Radar_RawTarget_Data_024  MsgIDType=Standard (11-bit identifier)  MsgIdentifier=1048  MsgLength=8  SignalInfo={'AZ_Winkel','22','10','LE','unsigned','Multiplexed','0','0.16','-81.76','-81.76','81.92';'EL_Angle','37','10','LE','unsigned','Multiplexed','1','0.04','-20.44','-20.44','20.48';'Internal_used','14','8','LE','unsigned','Multiplexed','0','1','0','-Inf','Inf';'Internal_used2','32','7','LE','unsigned','Multiplexed','0','1','0','-Inf','Inf';'Internal_used3','51','7','LE','unsigned','Multiplexed','0','1','0','-Inf','Inf';'Internal_used4','58','6','LE','unsigned','Multiplexed','0','1','0','-Inf','Inf';'Internal_used5','9','8','LE','unsigned','Multiplexed','1','1','0','-Inf','Inf';'Internal_used6','17','8','LE','unsigned','Multiplexed','1','1','0','-Inf','Inf';'Internal_used7','25','7','LE','unsigned','Multiplexed','1','1','0','-Inf','Inf';'Mode_Signal','0','1','LE','unsigned','Multiplexor','0','1','0','0','1';'RCS','1','7','LE','unsigned','Multiplexed','1','0.2','-15','-15','36';'Range1','1','13','LE','unsigned','Multiplexed','0','0.04','0','0','327.64';'Reserve_3','32','5','LE','unsigned','Multiplexed','1','1','0','-Inf','Inf';'Reserve_4','47','16','LE','unsigned','Multiplexed','1','1','0','-Inf','Inf';'Speed_Radial','39','12','LE','unsigned','Multiplexed','0','0.04','-119.68','-44.12','119.68'}  IDPort=on  TimestampPort=on  ErrorPort=off  RemotePort=off  LengthPort=off  StatusPort=off  ApplyMinMax=off
      settings: DataFormat=CANdb specified signals
  CAN Unpack26 : canmsglib/CAN Unpack  CANdbFile=eWolf_SensorCAN.dbc  MsgList=Radar_RawTarget_Data_025  MsgName=Radar_RawTarget_Data_025  MsgIDType=Standard (11-bit identifier)  MsgIdentifier=1049  MsgLength=8  SignalInfo={'AZ_Winkel','22','10','LE','unsigned','Multiplexed','0','0.16','-81.76','-81.76','81.92';'EL_Angle','37','10','LE','unsigned','Multiplexed','1','0.04','-20.44','-20.44','20.48';'Internal_used','14','8','LE','unsigned','Multiplexed','0','1','0','-Inf','Inf';'Internal_used2','32','7','LE','unsigned','Multiplexed','0','1','0','-Inf','Inf';'Internal_used3','51','7','LE','unsigned','Multiplexed','0','1','0','-Inf','Inf';'Internal_used4','58','6','LE','unsigned','Multiplexed','0','1','0','-Inf','Inf';'Internal_used5','9','8','LE','unsigned','Multiplexed','1','1','0','-Inf','Inf';'Internal_used6','17','8','LE','unsigned','Multiplexed','1','1','0','-Inf','Inf';'Internal_used7','25','7','LE','unsigned','Multiplexed','1','1','0','-Inf','Inf';'Mode_Signal','0','1','LE','unsigned','Multiplexor','0','1','0','0','1';'RCS','1','7','LE','unsigned','Multiplexed','1','0.2','-15','-15','36';'Range1','1','13','LE','unsigned','Multiplexed','0','0.04','0','0','327.64';'Reserve_3','32','5','LE','unsigned','Multiplexed','1','1','0','-Inf','Inf';'Reserve_4','47','16','LE','unsigned','Multiplexed','1','1','0','-Inf','Inf';'Speed_Radial','39','12','LE','unsigned','Multiplexed','0','0.04','-119.68','-44.12','119.68'}  IDPort=on  TimestampPort=on  ErrorPort=off  RemotePort=off  LengthPort=off  StatusPort=off  ApplyMinMax=off
      settings: DataFormat=CANdb specified signals
  CAN Unpack27 : canmsglib/CAN Unpack  CANdbFile=eWolf_SensorCAN.dbc  MsgList=Radar_RawTarget_Data_026  MsgName=Radar_RawTarget_Data_026  MsgIDType=Standard (11-bit identifier)  MsgIdentifier=1050  MsgLength=8  SignalInfo={'AZ_Winkel','22','10','LE','unsigned','Multiplexed','0','0.16','-81.76','-81.76','81.92';'EL_Angle','37','10','LE','unsigned','Multiplexed','1','0.04','-20.44','-20.44','20.48';'Internal_used','14','8','LE','unsigned','Multiplexed','0','1','0','-Inf','Inf';'Internal_used2','32','7','LE','unsigned','Multiplexed','0','1','0','-Inf','Inf';'Internal_used3','51','7','LE','unsigned','Multiplexed','0','1','0','-Inf','Inf';'Internal_used4','58','6','LE','unsigned','Multiplexed','0','1','0','-Inf','Inf';'Internal_used5','9','8','LE','unsigned','Multiplexed','1','1','0','-Inf','Inf';'Internal_used6','17','8','LE','unsigned','Multiplexed','1','1','0','-Inf','Inf';'Internal_used7','25','7','LE','unsigned','Multiplexed','1','1','0','-Inf','Inf';'Mode_Signal','0','1','LE','unsigned','Multiplexor','0','1','0','0','1';'RCS','1','7','LE','unsigned','Multiplexed','1','0.2','-15','-15','36';'Range1','1','13','LE','unsigned','Multiplexed','0','0.04','0','0','327.64';'Reserve_3','32','5','LE','unsigned','Multiplexed','1','1','0','-Inf','Inf';'Reserve_4','47','16','LE','unsigned','Multiplexed','1','1','0','-Inf','Inf';'Speed_Radial','39','12','LE','unsigned','Multiplexed','0','0.04','-119.68','-44.12','119.68'}  IDPort=on  TimestampPort=on  ErrorPort=off  RemotePort=off  LengthPort=off  StatusPort=off  ApplyMinMax=off
      settings: DataFormat=CANdb specified signals
  CAN Unpack28 : canmsglib/CAN Unpack  CANdbFile=eWolf_SensorCAN.dbc  MsgList=Radar_RawTarget_Data_027  MsgName=Radar_RawTarget_Data_027  MsgIDType=Standard (11-bit identifier)  MsgIdentifier=1051  MsgLength=8  SignalInfo={'AZ_Winkel','22','10','LE','unsigned','Multiplexed','0','0.16','-81.76','-81.76','81.92';'EL_Angle','37','10','LE','unsigned','Multiplexed','1','0.04','-20.44','-20.44','20.48';'Internal_used','14','8','LE','unsigned','Multiplexed','0','1','0','-Inf','Inf';'Internal_used2','32','7','LE','unsigned','Multiplexed','0','1','0','-Inf','Inf';'Internal_used3','51','7','LE','unsigned','Multiplexed','0','1','0','-Inf','Inf';'Internal_used4','58','6','LE','unsigned','Multiplexed','0','1','0','-Inf','Inf';'Internal_used5','9','8','LE','unsigned','Multiplexed','1','1','0','-Inf','Inf';'Internal_used6','17','8','LE','unsigned','Multiplexed','1','1','0','-Inf','Inf';'Internal_used7','25','7','LE','unsigned','Multiplexed','1','1','0','-Inf','Inf';'Mode_Signal','0','1','LE','unsigned','Multiplexor','0','1','0','0','1';'RCS','1','7','LE','unsigned','Multiplexed','1','0.2','-15','-15','36';'Range1','1','13','LE','unsigned','Multiplexed','0','0.04','0','0','327.64';'Reserve_3','32','5','LE','unsigned','Multiplexed','1','1','0','-Inf','Inf';'Reserve_4','47','16','LE','unsigned','Multiplexed','1','1','0','-Inf','Inf';'Speed_Radial','39','12','LE','unsigned','Multiplexed','0','0.04','-119.68','-44.12','119.68'}  IDPort=on  TimestampPort=on  ErrorPort=off  RemotePort=off  LengthPort=off  StatusPort=off  ApplyMinMax=off
      settings: DataFormat=CANdb specified signals
  CAN Unpack29 : canmsglib/CAN Unpack  CANdbFile=eWolf_SensorCAN.dbc  MsgList=Radar_RawTarget_Data_028  MsgName=Radar_RawTarget_Data_028  MsgIDType=Standard (11-bit identifier)  MsgIdentifier=1052  MsgLength=8  SignalInfo={'AZ_Winkel','22','10','LE','unsigned','Multiplexed','0','0.16','-81.76','-81.76','81.92';'EL_Angle','37','10','LE','unsigned','Multiplexed','1','0.04','-20.44','-20.44','20.48';'Internal_used','14','8','LE','unsigned','Multiplexed','0','1','0','-Inf','Inf';'Internal_used2','32','7','LE','unsigned','Multiplexed','0','1','0','-Inf','Inf';'Internal_used3','51','7','LE','unsigned','Multiplexed','0','1','0','-Inf','Inf';'Internal_used4','58','6','LE','unsigned','Multiplexed','0','1','0','-Inf','Inf';'Internal_used5','9','8','LE','unsigned','Multiplexed','1','1','0','-Inf','Inf';'Internal_used6','17','8','LE','unsigned','Multiplexed','1','1','0','-Inf','Inf';'Internal_used7','25','7','LE','unsigned','Multiplexed','1','1','0','-Inf','Inf';'Mode_Signal','0','1','LE','unsigned','Multiplexor','0','1','0','0','1';'RCS','1','7','LE','unsigned','Multiplexed','1','0.2','-15','-15','36';'Range1','1','13','LE','unsigned','Multiplexed','0','0.04','0','0','327.64';'Reserve_3','32','5','LE','unsigned','Multiplexed','1','1','0','-Inf','Inf';'Reserve_4','47','16','LE','unsigned','Multiplexed','1','1','0','-Inf','Inf';'Speed_Radial','39','12','LE','unsigned','Multiplexed','0','0.04','-119.68','-44.12','119.68'}  IDPort=on  TimestampPort=on  ErrorPort=off  RemotePort=off  LengthPort=off  StatusPort=off  ApplyMinMax=off
      settings: DataFormat=CANdb specified signals
  CAN Unpack3 : canmsglib/CAN Unpack  CANdbFile=eWolf_SensorCAN.dbc  MsgList=Radar_RawTarget_Data_001  MsgName=Radar_RawTarget_Data_001  MsgIDType=Standard (11-bit identifier)  MsgIdentifier=1025  MsgLength=8  SignalInfo={'AZ_Winkel','22','10','LE','unsigned','Multiplexed','0','0.16','-81.76','-81.76','81.92';'EL_Angle','37','10','LE','unsigned','Multiplexed','1','0.04','-20.44','-20.44','20.48';'Internal_used','14','8','LE','unsigned','Multiplexed','0','1','0','-Inf','Inf';'Internal_used2','32','7','LE','unsigned','Multiplexed','0','1','0','-Inf','Inf';'Internal_used3','51','7','LE','unsigned','Multiplexed','0','1','0','-Inf','Inf';'Internal_used4','58','6','LE','unsigned','Multiplexed','0','1','0','-Inf','Inf';'Internal_used5','9','8','LE','unsigned','Multiplexed','1','1','0','-Inf','Inf';'Internal_used6','17','8','LE','unsigned','Multiplexed','1','1','0','-Inf','Inf';'Internal_used7','25','7','LE','unsigned','Multiplexed','1','1','0','-Inf','Inf';'Mode_Signal','0','1','LE','unsigned','Multiplexor','0','1','0','0','1';'RCS','1','7','LE','unsigned','Multiplexed','1','0.2','-15','-15','36';'Range1','1','13','LE','unsigned','Multiplexed','0','0.04','0','0','327.64';'Reserve_3','32','5','LE','unsigned','Multiplexed','1','1','0','-Inf','Inf';'Reserve_4','47','16','LE','unsigned','Multiplexed','1','1','0','-Inf','Inf';'Speed_Radial','39','12','LE','unsigned','Multiplexed','0','0.04','-119.68','-44.12','119.68'}  IDPort=on  TimestampPort=on  ErrorPort=off  RemotePort=off  LengthPort=off  StatusPort=off  ApplyMinMax=off
      settings: DataFormat=CANdb specified signals
  CAN Unpack30 : canmsglib/CAN Unpack  CANdbFile=eWolf_SensorCAN.dbc  MsgList=Radar_RawTarget_Data_029  MsgName=Radar_RawTarget_Data_029  MsgIDType=Standard (11-bit identifier)  MsgIdentifier=1053  MsgLength=8  SignalInfo={'AZ_Winkel','22','10','LE','unsigned','Multiplexed','0','0.16','-81.76','-81.76','81.92';'EL_Angle','37','10','LE','unsigned','Multiplexed','1','0.04','-20.44','-20.44','20.48';'Internal_used','14','8','LE','unsigned','Multiplexed','0','1','0','-Inf','Inf';'Internal_used2','32','7','LE','unsigned','Multiplexed','0','1','0','-Inf','Inf';'Internal_used3','51','7','LE','unsigned','Multiplexed','0','1','0','-Inf','Inf';'Internal_used4','58','6','LE','unsigned','Multiplexed','0','1','0','-Inf','Inf';'Internal_used5','9','8','LE','unsigned','Multiplexed','1','1','0','-Inf','Inf';'Internal_used6','17','8','LE','unsigned','Multiplexed','1','1','0','-Inf','Inf';'Internal_used7','25','7','LE','unsigned','Multiplexed','1','1','0','-Inf','Inf';'Mode_Signal','0','1','LE','unsigned','Multiplexor','0','1','0','0','1';'RCS','1','7','LE','unsigned','Multiplexed','1','0.2','-15','-15','36';'Range1','1','13','LE','unsigned','Multiplexed','0','0.04','0','0','327.64';'Reserve_3','32','5','LE','unsigned','Multiplexed','1','1','0','-Inf','Inf';'Reserve_4','47','16','LE','unsigned','Multiplexed','1','1','0','-Inf','Inf';'Speed_Radial','39','12','LE','unsigned','Multiplexed','0','0.04','-119.68','-44.12','119.68'}  IDPort=on  TimestampPort=on  ErrorPort=off  RemotePort=off  LengthPort=off  StatusPort=off  ApplyMinMax=off
      settings: DataFormat=CANdb specified signals
  CAN Unpack31 : canmsglib/CAN Unpack  CANdbFile=eWolf_SensorCAN.dbc  MsgList=Radar_RawTarget_Data_030  MsgName=Radar_RawTarget_Data_030  MsgIDType=Standard (11-bit identifier)  MsgIdentifier=1054  MsgLength=8  SignalInfo={'AZ_Winkel','22','10','LE','unsigned','Multiplexed','0','0.16','-81.76','-81.76','81.92';'EL_Angle','37','10','LE','unsigned','Multiplexed','1','0.04','-20.44','-20.44','20.48';'Internal_used','14','8','LE','unsigned','Multiplexed','0','1','0','-Inf','Inf';'Internal_used2','32','7','LE','unsigned','Multiplexed','0','1','0','-Inf','Inf';'Internal_used3','51','7','LE','unsigned','Multiplexed','0','1','0','-Inf','Inf';'Internal_used4','58','6','LE','unsigned','Multiplexed','0','1','0','-Inf','Inf';'Internal_used5','9','8','LE','unsigned','Multiplexed','1','1','0','-Inf','Inf';'Internal_used6','17','8','LE','unsigned','Multiplexed','1','1','0','-Inf','Inf';'Internal_used7','25','7','LE','unsigned','Multiplexed','1','1','0','-Inf','Inf';'Mode_Signal','0','1','LE','unsigned','Multiplexor','0','1','0','0','1';'RCS','1','7','LE','unsigned','Multiplexed','1','0.2','-15','-15','36';'Range1','1','13','LE','unsigned','Multiplexed','0','0.04','0','0','327.64';'Reserve_3','32','5','LE','unsigned','Multiplexed','1','1','0','-Inf','Inf';'Reserve_4','47','16','LE','unsigned','Multiplexed','1','1','0','-Inf','Inf';'Speed_Radial','39','12','LE','unsigned','Multiplexed','0','0.04','-119.68','-44.12','119.68'}  IDPort=on  TimestampPort=on  ErrorPort=off  RemotePort=off  LengthPort=off  StatusPort=off  ApplyMinMax=off
      settings: DataFormat=CANdb specified signals
  CAN Unpack32 : canmsglib/CAN Unpack  CANdbFile=eWolf_SensorCAN.dbc  MsgList=Radar_RawTarget_Data_031  MsgName=Radar_RawTarget_Data_031  MsgIDType=Standard (11-bit identifier)  MsgIdentifier=1055  MsgLength=8  SignalInfo={'AZ_Winkel','22','10','LE','unsigned','Multiplexed','0','0.16','-81.76','-81.76','81.92';'EL_Angle','37','10','LE','unsigned','Multiplexed','1','0.04','-20.44','-20.44','20.48';'Internal_used','14','8','LE','unsigned','Multiplexed','0','1','0','-Inf','Inf';'Internal_used2','32','7','LE','unsigned','Multiplexed','0','1','0','-Inf','Inf';'Internal_used3','51','7','LE','unsigned','Multiplexed','0','1','0','-Inf','Inf';'Internal_used4','58','6','LE','unsigned','Multiplexed','0','1','0','-Inf','Inf';'Internal_used5','9','8','LE','unsigned','Multiplexed','1','1','0','-Inf','Inf';'Internal_used6','17','8','LE','unsigned','Multiplexed','1','1','0','-Inf','Inf';'Internal_used7','25','7','LE','unsigned','Multiplexed','1','1','0','-Inf','Inf';'Mode_Signal','0','1','LE','unsigned','Multiplexor','0','1','0','0','1';'RCS','1','7','LE','unsigned','Multiplexed','1','0.2','-15','-15','36';'Range1','1','13','LE','unsigned','Multiplexed','0','0.04','0','0','327.64';'Reserve_3','32','5','LE','unsigned','Multiplexed','1','1','0','-Inf','Inf';'Reserve_4','47','16','LE','unsigned','Multiplexed','1','1','0','-Inf','Inf';'Speed_Radial','39','12','LE','unsigned','Multiplexed','0','0.04','-119.68','-44.12','119.68'}  IDPort=on  TimestampPort=on  ErrorPort=off  RemotePort=off  LengthPort=off  StatusPort=off  ApplyMinMax=off
      settings: DataFormat=CANdb specified signals
  CAN Unpack33 : canmsglib/CAN Unpack  CANdbFile=eWolf_SensorCAN.dbc  MsgList=Radar_RawTarget_Data_032  MsgName=Radar_RawTarget_Data_032  MsgIDType=Standard (11-bit identifier)  MsgIdentifier=1056  MsgLength=8  SignalInfo={'AZ_Winkel','22','10','LE','unsigned','Multiplexed','0','0.16','-81.76','-81.76','81.92';'EL_Angle','37','10','LE','unsigned','Multiplexed','1','0.04','-20.44','-20.44','20.48';'Internal_used','14','8','LE','unsigned','Multiplexed','0','1','0','-Inf','Inf';'Internal_used2','32','7','LE','unsigned','Multiplexed','0','1','0','-Inf','Inf';'Internal_used3','51','7','LE','unsigned','Multiplexed','0','1','0','-Inf','Inf';'Internal_used4','58','6','LE','unsigned','Multiplexed','0','1','0','-Inf','Inf';'Internal_used5','9','8','LE','unsigned','Multiplexed','1','1','0','-Inf','Inf';'Internal_used6','17','8','LE','unsigned','Multiplexed','1','1','0','-Inf','Inf';'Internal_used7','25','7','LE','unsigned','Multiplexed','1','1','0','-Inf','Inf';'Mode_Signal','0','1','LE','unsigned','Multiplexor','0','1','0','0','1';'RCS','1','7','LE','unsigned','Multiplexed','1','0.2','-15','-15','36';'Range1','1','13','LE','unsigned','Multiplexed','0','0.04','0','0','327.64';'Reserve_3','32','5','LE','unsigned','Multiplexed','1','1','0','-Inf','Inf';'Reserve_4','47','16','LE','unsigned','Multiplexed','1','1','0','-Inf','Inf';'Speed_Radial','39','12','LE','unsigned','Multiplexed','0','0.04','-119.68','-44.12','119.68'}  IDPort=on  TimestampPort=on  ErrorPort=off  RemotePort=off  LengthPort=off  StatusPort=off  ApplyMinMax=off
      settings: DataFormat=CANdb specified signals
  CAN Unpack34 : canmsglib/CAN Unpack  CANdbFile=eWolf_SensorCAN.dbc  MsgList=Radar_RawTarget_Data_033  MsgName=Radar_RawTarget_Data_033  MsgIDType=Standard (11-bit identifier)  MsgIdentifier=1057  MsgLength=8  SignalInfo={'AZ_Winkel','22','10','LE','unsigned','Multiplexed','0','0.16','-81.76','-81.76','81.92';'EL_Angle','37','10','LE','unsigned','Multiplexed','1','0.04','-20.44','-20.44','20.48';'Internal_used','14','8','LE','unsigned','Multiplexed','0','1','0','-Inf','Inf';'Internal_used2','32','7','LE','unsigned','Multiplexed','0','1','0','-Inf','Inf';'Internal_used3','51','7','LE','unsigned','Multiplexed','0','1','0','-Inf','Inf';'Internal_used4','58','6','LE','unsigned','Multiplexed','0','1','0','-Inf','Inf';'Internal_used5','9','8','LE','unsigned','Multiplexed','1','1','0','-Inf','Inf';'Internal_used6','17','8','LE','unsigned','Multiplexed','1','1','0','-Inf','Inf';'Internal_used7','25','7','LE','unsigned','Multiplexed','1','1','0','-Inf','Inf';'Mode_Signal','0','1','LE','unsigned','Multiplexor','0','1','0','0','1';'RCS','1','7','LE','unsigned','Multiplexed','1','0.2','-15','-15','36';'Range1','1','13','LE','unsigned','Multiplexed','0','0.04','0','0','327.64';'Reserve_3','32','5','LE','unsigned','Multiplexed','1','1','0','-Inf','Inf';'Reserve_4','47','16','LE','unsigned','Multiplexed','1','1','0','-Inf','Inf';'Speed_Radial','39','12','LE','unsigned','Multiplexed','0','0.04','-119.68','-44.12','119.68'}  IDPort=on  TimestampPort=on  ErrorPort=off  RemotePort=off  LengthPort=off  StatusPort=off  ApplyMinMax=off
      settings: DataFormat=CANdb specified signals
  CAN Unpack35 : canmsglib/CAN Unpack  CANdbFile=eWolf_SensorCAN.dbc  MsgList=Radar_RawTarget_Data_034  MsgName=Radar_RawTarget_Data_034  MsgIDType=Standard (11-bit identifier)  MsgIdentifier=1058  MsgLength=8  SignalInfo={'AZ_Winkel','22','10','LE','unsigned','Multiplexed','0','0.16','-81.76','-81.76','81.92';'EL_Angle','37','10','LE','unsigned','Multiplexed','1','0.04','-20.44','-20.44','20.48';'Internal_used','14','8','LE','unsigned','Multiplexed','0','1','0','-Inf','Inf';'Internal_used2','32','7','LE','unsigned','Multiplexed','0','1','0','-Inf','Inf';'Internal_used3','51','7','LE','unsigned','Multiplexed','0','1','0','-Inf','Inf';'Internal_used4','58','6','LE','unsigned','Multiplexed','0','1','0','-Inf','Inf';'Internal_used5','9','8','LE','unsigned','Multiplexed','1','1','0','-Inf','Inf';'Internal_used6','17','8','LE','unsigned','Multiplexed','1','1','0','-Inf','Inf';'Internal_used7','25','7','LE','unsigned','Multiplexed','1','1','0','-Inf','Inf';'Mode_Signal','0','1','LE','unsigned','Multiplexor','0','1','0','0','1';'RCS','1','7','LE','unsigned','Multiplexed','1','0.2','-15','-15','36';'Range1','1','13','LE','unsigned','Multiplexed','0','0.04','0','0','327.64';'Reserve_3','32','5','LE','unsigned','Multiplexed','1','1','0','-Inf','Inf';'Reserve_4','47','16','LE','unsigned','Multiplexed','1','1','0','-Inf','Inf';'Speed_Radial','39','12','LE','unsigned','Multiplexed','0','0.04','-119.68','-44.12','119.68'}  IDPort=on  TimestampPort=on  ErrorPort=off  RemotePort=off  LengthPort=off  StatusPort=off  ApplyMinMax=off
      settings: DataFormat=CANdb specified signals
  CAN Unpack36 : canmsglib/CAN Unpack  CANdbFile=eWolf_SensorCAN.dbc  MsgList=Radar_RawTarget_Data_035  MsgName=Radar_RawTarget_Data_035  MsgIDType=Standard (11-bit identifier)  MsgIdentifier=1059  MsgLength=8  SignalInfo={'AZ_Winkel','22','10','LE','unsigned','Multiplexed','0','0.16','-81.76','-81.76','81.92';'EL_Angle','37','10','LE','unsigned','Multiplexed','1','0.04','-20.44','-20.44','20.48';'Internal_used','14','8','LE','unsigned','Multiplexed','0','1','0','-Inf','Inf';'Internal_used2','32','7','LE','unsigned','Multiplexed','0','1','0','-Inf','Inf';'Internal_used3','51','7','LE','unsigned','Multiplexed','0','1','0','-Inf','Inf';'Internal_used4','58','6','LE','unsigned','Multiplexed','0','1','0','-Inf','Inf';'Internal_used5','9','8','LE','unsigned','Multiplexed','1','1','0','-Inf','Inf';'Internal_used6','17','8','LE','unsigned','Multiplexed','1','1','0','-Inf','Inf';'Internal_used7','25','7','LE','unsigned','Multiplexed','1','1','0','-Inf','Inf';'Mode_Signal','0','1','LE','unsigned','Multiplexor','0','1','0','0','1';'RCS','1','7','LE','unsigned','Multiplexed','1','0.2','-15','-15','36';'Range1','1','13','LE','unsigned','Multiplexed','0','0.04','0','0','327.64';'Reserve_3','32','5','LE','unsigned','Multiplexed','1','1','0','-Inf','Inf';'Reserve_4','47','16','LE','unsigned','Multiplexed','1','1','0','-Inf','Inf';'Speed_Radial','39','12','LE','unsigned','Multiplexed','0','0.04','-119.68','-44.12','119.68'}  IDPort=on  TimestampPort=on  ErrorPort=off  RemotePort=off  LengthPort=off  StatusPort=off  ApplyMinMax=off
      settings: DataFormat=CANdb specified signals
  CAN Unpack37 : canmsglib/CAN Unpack  CANdbFile=eWolf_SensorCAN.dbc  MsgList=Radar_RawTarget_Data_036  MsgName=Radar_RawTarget_Data_036  MsgIDType=Standard (11-bit identifier)  MsgIdentifier=1060  MsgLength=8  SignalInfo={'AZ_Winkel','22','10','LE','unsigned','Multiplexed','0','0.16','-81.76','-81.76','81.92';'EL_Angle','37','10','LE','unsigned','Multiplexed','1','0.04','-20.44','-20.44','20.48';'Internal_used','14','8','LE','unsigned','Multiplexed','0','1','0','-Inf','Inf';'Internal_used2','32','7','LE','unsigned','Multiplexed','0','1','0','-Inf','Inf';'Internal_used3','51','7','LE','unsigned','Multiplexed','0','1','0','-Inf','Inf';'Internal_used4','58','6','LE','unsigned','Multiplexed','0','1','0','-Inf','Inf';'Internal_used5','9','8','LE','unsigned','Multiplexed','1','1','0','-Inf','Inf';'Internal_used6','17','8','LE','unsigned','Multiplexed','1','1','0','-Inf','Inf';'Internal_used7','25','7','LE','unsigned','Multiplexed','1','1','0','-Inf','Inf';'Mode_Signal','0','1','LE','unsigned','Multiplexor','0','1','0','0','1';'RCS','1','7','LE','unsigned','Multiplexed','1','0.2','-15','-15','36';'Range1','1','13','LE','unsigned','Multiplexed','0','0.04','0','0','327.64';'Reserve_3','32','5','LE','unsigned','Multiplexed','1','1','0','-Inf','Inf';'Reserve_4','47','16','LE','unsigned','Multiplexed','1','1','0','-Inf','Inf';'Speed_Radial','39','12','LE','unsigned','Multiplexed','0','0.04','-119.68','-44.12','119.68'}  IDPort=on  TimestampPort=on  ErrorPort=off  RemotePort=off  LengthPort=off  StatusPort=off  ApplyMinMax=off
      settings: DataFormat=CANdb specified signals
  CAN Unpack38 : canmsglib/CAN Unpack  CANdbFile=eWolf_SensorCAN.dbc  MsgList=Radar_RawTarget_Data_037  MsgName=Radar_RawTarget_Data_037  MsgIDType=Standard (11-bit identifier)  MsgIdentifier=1061  MsgLength=8  SignalInfo={'AZ_Winkel','22','10','LE','unsigned','Multiplexed','0','0.16','-81.76','-81.76','81.92';'EL_Angle','37','10','LE','unsigned','Multiplexed','1','0.04','-20.44','-20.44','20.48';'Internal_used','14','8','LE','unsigned','Multiplexed','0','1','0','-Inf','Inf';'Internal_used2','32','7','LE','unsigned','Multiplexed','0','1','0','-Inf','Inf';'Internal_used3','51','7','LE','unsigned','Multiplexed','0','1','0','-Inf','Inf';'Internal_used4','58','6','LE','unsigned','Multiplexed','0','1','0','-Inf','Inf';'Internal_used5','9','8','LE','unsigned','Multiplexed','1','1','0','-Inf','Inf';'Internal_used6','17','8','LE','unsigned','Multiplexed','1','1','0','-Inf','Inf';'Internal_used7','25','7','LE','unsigned','Multiplexed','1','1','0','-Inf','Inf';'Mode_Signal','0','1','LE','unsigned','Multiplexor','0','1','0','0','1';'RCS','1','7','LE','unsigned','Multiplexed','1','0.2','-15','-15','36';'Range1','1','13','LE','unsigned','Multiplexed','0','0.04','0','0','327.64';'Reserve_3','32','5','LE','unsigned','Multiplexed','1','1','0','-Inf','Inf';'Reserve_4','47','16','LE','unsigned','Multiplexed','1','1','0','-Inf','Inf';'Speed_Radial','39','12','LE','unsigned','Multiplexed','0','0.04','-119.68','-44.12','119.68'}  IDPort=on  TimestampPort=on  ErrorPort=off  RemotePort=off  LengthPort=off  StatusPort=off  ApplyMinMax=off
      settings: DataFormat=CANdb specified signals
  CAN Unpack39 : canmsglib/CAN Unpack  CANdbFile=eWolf_SensorCAN.dbc  MsgList=Radar_RawTarget_Data_038  MsgName=Radar_RawTarget_Data_038  MsgIDType=Standard (11-bit identifier)  MsgIdentifier=1062  MsgLength=8  SignalInfo={'AZ_Winkel','22','10','LE','unsigned','Multiplexed','0','0.16','-81.76','-81.76','81.92';'EL_Angle','37','10','LE','unsigned','Multiplexed','1','0.04','-20.44','-20.44','20.48';'Internal_used','14','8','LE','unsigned','Multiplexed','0','1','0','-Inf','Inf';'Internal_used2','32','7','LE','unsigned','Multiplexed','0','1','0','-Inf','Inf';'Internal_used3','51','7','LE','unsigned','Multiplexed','0','1','0','-Inf','Inf';'Internal_used4','58','6','LE','unsigned','Multiplexed','0','1','0','-Inf','Inf';'Internal_used5','9','8','LE','unsigned','Multiplexed','1','1','0','-Inf','Inf';'Internal_used6','17','8','LE','unsigned','Multiplexed','1','1','0','-Inf','Inf';'Internal_used7','25','7','LE','unsigned','Multiplexed','1','1','0','-Inf','Inf';'Mode_Signal','0','1','LE','unsigned','Multiplexor','0','1','0','0','1';'RCS','1','7','LE','unsigned','Multiplexed','1','0.2','-15','-15','36';'Range1','1','13','LE','unsigned','Multiplexed','0','0.04','0','0','327.64';'Reserve_3','32','5','LE','unsigned','Multiplexed','1','1','0','-Inf','Inf';'Reserve_4','47','16','LE','unsigned','Multiplexed','1','1','0','-Inf','Inf';'Speed_Radial','39','12','LE','unsigned','Multiplexed','0','0.04','-119.68','-44.12','119.68'}  IDPort=on  TimestampPort=on  ErrorPort=off  RemotePort=off  LengthPort=off  StatusPort=off  ApplyMinMax=off
      settings: DataFormat=CANdb specified signals
  CAN Unpack4 : canmsglib/CAN Unpack  CANdbFile=eWolf_SensorCAN.dbc  MsgList=Radar_RawTarget_Data_003  MsgName=Radar_RawTarget_Data_003  MsgIDType=Standard (11-bit identifier)  MsgIdentifier=1027  MsgLength=8  SignalInfo={'AZ_Winkel','22','10','LE','unsigned','Multiplexed','0','0.16','-81.76','-81.76','81.92';'EL_Angle','37','10','LE','unsigned','Multiplexed','1','0.04','-20.44','-20.44','20.48';'Internal_used','14','8','LE','unsigned','Multiplexed','0','1','0','-Inf','Inf';'Internal_used2','32','7','LE','unsigned','Multiplexed','0','1','0','-Inf','Inf';'Internal_used3','51','7','LE','unsigned','Multiplexed','0','1','0','-Inf','Inf';'Internal_used4','58','6','LE','unsigned','Multiplexed','0','1','0','-Inf','Inf';'Internal_used5','9','8','LE','unsigned','Multiplexed','1','1','0','-Inf','Inf';'Internal_used6','17','8','LE','unsigned','Multiplexed','1','1','0','-Inf','Inf';'Internal_used7','25','7','LE','unsigned','Multiplexed','1','1','0','-Inf','Inf';'Mode_Signal','0','1','LE','unsigned','Multiplexor','0','1','0','0','1';'RCS','1','7','LE','unsigned','Multiplexed','1','0.2','-15','-15','36';'Range1','1','13','LE','unsigned','Multiplexed','0','0.04','0','0','327.64';'Reserve_3','32','5','LE','unsigned','Multiplexed','1','1','0','-Inf','Inf';'Reserve_4','47','16','LE','unsigned','Multiplexed','1','1','0','-Inf','Inf';'Speed_Radial','39','12','LE','unsigned','Multiplexed','0','0.04','-119.68','-44.12','119.68'}  IDPort=on  TimestampPort=on  ErrorPort=off  RemotePort=off  LengthPort=off  StatusPort=off  ApplyMinMax=off
      settings: DataFormat=CANdb specified signals
  CAN Unpack40 : canmsglib/CAN Unpack  CANdbFile=eWolf_SensorCAN.dbc  MsgList=Radar_RawTarget_Data_039  MsgName=Radar_RawTarget_Data_039  MsgIDType=Standard (11-bit identifier)  MsgIdentifier=1063  MsgLength=8  SignalInfo={'AZ_Winkel','22','10','LE','unsigned','Multiplexed','0','0.16','-81.76','-81.76','81.92';'EL_Angle','37','10','LE','unsigned','Multiplexed','1','0.04','-20.44','-20.44','20.48';'Internal_used','14','8','LE','unsigned','Multiplexed','0','1','0','-Inf','Inf';'Internal_used2','32','7','LE','unsigned','Multiplexed','0','1','0','-Inf','Inf';'Internal_used3','51','7','LE','unsigned','Multiplexed','0','1','0','-Inf','Inf';'Internal_used4','58','6','LE','unsigned','Multiplexed','0','1','0','-Inf','Inf';'Internal_used5','9','8','LE','unsigned','Multiplexed','1','1','0','-Inf','Inf';'Internal_used6','17','8','LE','unsigned','Multiplexed','1','1','0','-Inf','Inf';'Internal_used7','25','7','LE','unsigned','Multiplexed','1','1','0','-Inf','Inf';'Mode_Signal','0','1','LE','unsigned','Multiplexor','0','1','0','0','1';'RCS','1','7','LE','unsigned','Multiplexed','1','0.2','-15','-15','36';'Range1','1','13','LE','unsigned','Multiplexed','0','0.04','0','0','327.64';'Reserve_3','32','5','LE','unsigned','Multiplexed','1','1','0','-Inf','Inf';'Reserve_4','47','16','LE','unsigned','Multiplexed','1','1','0','-Inf','Inf';'Speed_Radial','39','12','LE','unsigned','Multiplexed','0','0.04','-119.68','-44.12','119.68'}  IDPort=on  TimestampPort=on  ErrorPort=off  RemotePort=off  LengthPort=off  StatusPort=off  ApplyMinMax=off
      settings: DataFormat=CANdb specified signals
  CAN Unpack41 : canmsglib/CAN Unpack  CANdbFile=eWolf_SensorCAN.dbc  MsgList=Radar_RawTarget_Data_040  MsgName=Radar_RawTarget_Data_040  MsgIDType=Standard (11-bit identifier)  MsgIdentifier=1064  MsgLength=8  SignalInfo={'AZ_Winkel','22','10','LE','unsigned','Multiplexed','0','0.16','-81.76','-81.76','81.92';'EL_Angle','37','10','LE','unsigned','Multiplexed','1','0.04','-20.44','-20.44','20.48';'Internal_used','14','8','LE','unsigned','Multiplexed','0','1','0','-Inf','Inf';'Internal_used2','32','7','LE','unsigned','Multiplexed','0','1','0','-Inf','Inf';'Internal_used3','51','7','LE','unsigned','Multiplexed','0','1','0','-Inf','Inf';'Internal_used4','58','6','LE','unsigned','Multiplexed','0','1','0','-Inf','Inf';'Internal_used5','9','8','LE','unsigned','Multiplexed','1','1','0','-Inf','Inf';'Internal_used6','17','8','LE','unsigned','Multiplexed','1','1','0','-Inf','Inf';'Internal_used7','25','7','LE','unsigned','Multiplexed','1','1','0','-Inf','Inf';'Mode_Signal','0','1','LE','unsigned','Multiplexor','0','1','0','0','1';'RCS','1','7','LE','unsigned','Multiplexed','1','0.2','-15','-15','36';'Range1','1','13','LE','unsigned','Multiplexed','0','0.04','0','0','327.64';'Reserve_3','32','5','LE','unsigned','Multiplexed','1','1','0','-Inf','Inf';'Reserve_4','47','16','LE','unsigned','Multiplexed','1','1','0','-Inf','Inf';'Speed_Radial','39','12','LE','unsigned','Multiplexed','0','0.04','-119.68','-44.12','119.68'}  IDPort=on  TimestampPort=on  ErrorPort=off  RemotePort=off  LengthPort=off  StatusPort=off  ApplyMinMax=off
      settings: DataFormat=CANdb specified signals
  CAN Unpack42 : canmsglib/CAN Unpack  CANdbFile=eWolf_SensorCAN.dbc  MsgList=Radar_RawTarget_Data_041  MsgName=Radar_RawTarget_Data_041  MsgIDType=Standard (11-bit identifier)  MsgIdentifier=1065  MsgLength=8  SignalInfo={'AZ_Winkel','22','10','LE','unsigned','Multiplexed','0','0.16','-81.76','-81.76','81.92';'EL_Angle','37','10','LE','unsigned','Multiplexed','1','0.04','-20.44','-20.44','20.48';'Internal_used','14','8','LE','unsigned','Multiplexed','0','1','0','-Inf','Inf';'Internal_used2','32','7','LE','unsigned','Multiplexed','0','1','0','-Inf','Inf';'Internal_used3','51','7','LE','unsigned','Multiplexed','0','1','0','-Inf','Inf';'Internal_used4','58','6','LE','unsigned','Multiplexed','0','1','0','-Inf','Inf';'Internal_used5','9','8','LE','unsigned','Multiplexed','1','1','0','-Inf','Inf';'Internal_used6','17','8','LE','unsigned','Multiplexed','1','1','0','-Inf','Inf';'Internal_used7','25','7','LE','unsigned','Multiplexed','1','1','0','-Inf','Inf';'Mode_Signal','0','1','LE','unsigned','Multiplexor','0','1','0','0','1';'RCS','1','7','LE','unsigned','Multiplexed','1','0.2','-15','-15','36';'Range1','1','13','LE','unsigned','Multiplexed','0','0.04','0','0','327.64';'Reserve_3','32','5','LE','unsigned','Multiplexed','1','1','0','-Inf','Inf';'Reserve_4','47','16','LE','unsigned','Multiplexed','1','1','0','-Inf','Inf';'Speed_Radial','39','12','LE','unsigned','Multiplexed','0','0.04','-119.68','-44.12','119.68'}  IDPort=on  TimestampPort=on  ErrorPort=off  RemotePort=off  LengthPort=off  StatusPort=off  ApplyMinMax=off
      settings: DataFormat=CANdb specified signals
  CAN Unpack43 : canmsglib/CAN Unpack  CANdbFile=eWolf_SensorCAN.dbc  MsgList=Radar_RawTarget_Data_042  MsgName=Radar_RawTarget_Data_042  MsgIDType=Standard (11-bit identifier)  MsgIdentifier=1066  MsgLength=8  SignalInfo={'AZ_Winkel','22','10','LE','unsigned','Multiplexed','0','0.16','-81.76','-81.76','81.92';'EL_Angle','37','10','LE','unsigned','Multiplexed','1','0.04','-20.44','-20.44','20.48';'Internal_used','14','8','LE','unsigned','Multiplexed','0','1','0','-Inf','Inf';'Internal_used2','32','7','LE','unsigned','Multiplexed','0','1','0','-Inf','Inf';'Internal_used3','51','7','LE','unsigned','Multiplexed','0','1','0','-Inf','Inf';'Internal_used4','58','6','LE','unsigned','Multiplexed','0','1','0','-Inf','Inf';'Internal_used5','9','8','LE','unsigned','Multiplexed','1','1','0','-Inf','Inf';'Internal_used6','17','8','LE','unsigned','Multiplexed','1','1','0','-Inf','Inf';'Internal_used7','25','7','LE','unsigned','Multiplexed','1','1','0','-Inf','Inf';'Mode_Signal','0','1','LE','unsigned','Multiplexor','0','1','0','0','1';'RCS','1','7','LE','unsigned','Multiplexed','1','0.2','-15','-15','36';'Range1','1','13','LE','unsigned','Multiplexed','0','0.04','0','0','327.64';'Reserve_3','32','5','LE','unsigned','Multiplexed','1','1','0','-Inf','Inf';'Reserve_4','47','16','LE','unsigned','Multiplexed','1','1','0','-Inf','Inf';'Speed_Radial','39','12','LE','unsigned','Multiplexed','0','0.04','-119.68','-44.12','119.68'}  IDPort=on  TimestampPort=on  ErrorPort=off  RemotePort=off  LengthPort=off  StatusPort=off  ApplyMinMax=off
      settings: DataFormat=CANdb specified signals
  CAN Unpack44 : canmsglib/CAN Unpack  CANdbFile=eWolf_SensorCAN.dbc  MsgList=Radar_RawTarget_Data_043  MsgName=Radar_RawTarget_Data_043  MsgIDType=Standard (11-bit identifier)  MsgIdentifier=1067  MsgLength=8  SignalInfo={'AZ_Winkel','22','10','LE','unsigned','Multiplexed','0','0.16','-81.76','-81.76','81.92';'EL_Angle','37','10','LE','unsigned','Multiplexed','1','0.04','-20.44','-20.44','20.48';'Internal_used','14','8','LE','unsigned','Multiplexed','0','1','0','-Inf','Inf';'Internal_used2','32','7','LE','unsigned','Multiplexed','0','1','0','-Inf','Inf';'Internal_used3','51','7','LE','unsigned','Multiplexed','0','1','0','-Inf','Inf';'Internal_used4','58','6','LE','unsigned','Multiplexed','0','1','0','-Inf','Inf';'Internal_used5','9','8','LE','unsigned','Multiplexed','1','1','0','-Inf','Inf';'Internal_used6','17','8','LE','unsigned','Multiplexed','1','1','0','-Inf','Inf';'Internal_used7','25','7','LE','unsigned','Multiplexed','1','1','0','-Inf','Inf';'Mode_Signal','0','1','LE','unsigned','Multiplexor','0','1','0','0','1';'RCS','1','7','LE','unsigned','Multiplexed','1','0.2','-15','-15','36';'Range1','1','13','LE','unsigned','Multiplexed','0','0.04','0','0','327.64';'Reserve_3','32','5','LE','unsigned','Multiplexed','1','1','0','-Inf','Inf';'Reserve_4','47','16','LE','unsigned','Multiplexed','1','1','0','-Inf','Inf';'Speed_Radial','39','12','LE','unsigned','Multiplexed','0','0.04','-119.68','-44.12','119.68'}  IDPort=on  TimestampPort=on  ErrorPort=off  RemotePort=off  LengthPort=off  StatusPort=off  ApplyMinMax=off
      settings: DataFormat=CANdb specified signals
  CAN Unpack45 : canmsglib/CAN Unpack  CANdbFile=eWolf_SensorCAN.dbc  MsgList=Radar_RawTarget_Data_044  MsgName=Radar_RawTarget_Data_044  MsgIDType=Standard (11-bit identifier)  MsgIdentifier=1068  MsgLength=8  SignalInfo={'AZ_Winkel','22','10','LE','unsigned','Multiplexed','0','0.16','-81.76','-81.76','81.92';'EL_Angle','37','10','LE','unsigned','Multiplexed','1','0.04','-20.44','-20.44','20.48';'Internal_used','14','8','LE','unsigned','Multiplexed','0','1','0','-Inf','Inf';'Internal_used2','32','7','LE','unsigned','Multiplexed','0','1','0','-Inf','Inf';'Internal_used3','51','7','LE','unsigned','Multiplexed','0','1','0','-Inf','Inf';'Internal_used4','58','6','LE','unsigned','Multiplexed','0','1','0','-Inf','Inf';'Internal_used5','9','8','LE','unsigned','Multiplexed','1','1','0','-Inf','Inf';'Internal_used6','17','8','LE','unsigned','Multiplexed','1','1','0','-Inf','Inf';'Internal_used7','25','7','LE','unsigned','Multiplexed','1','1','0','-Inf','Inf';'Mode_Signal','0','1','LE','unsigned','Multiplexor','0','1','0','0','1';'RCS','1','7','LE','unsigned','Multiplexed','1','0.2','-15','-15','36';'Range1','1','13','LE','unsigned','Multiplexed','0','0.04','0','0','327.64';'Reserve_3','32','5','LE','unsigned','Multiplexed','1','1','0','-Inf','Inf';'Reserve_4','47','16','LE','unsigned','Multiplexed','1','1','0','-Inf','Inf';'Speed_Radial','39','12','LE','unsigned','Multiplexed','0','0.04','-119.68','-44.12','119.68'}  IDPort=on  TimestampPort=on  ErrorPort=off  RemotePort=off  LengthPort=off  StatusPort=off  ApplyMinMax=off
      settings: DataFormat=CANdb specified signals
  CAN Unpack46 : canmsglib/CAN Unpack  CANdbFile=eWolf_SensorCAN.dbc  MsgList=Radar_RawTarget_Data_045  MsgName=Radar_RawTarget_Data_045  MsgIDType=Standard (11-bit identifier)  MsgIdentifier=1069  MsgLength=8  SignalInfo={'AZ_Winkel','22','10','LE','unsigned','Multiplexed','0','0.16','-81.76','-81.76','81.92';'EL_Angle','37','10','LE','unsigned','Multiplexed','1','0.04','-20.44','-20.44','20.48';'Internal_used','14','8','LE','unsigned','Multiplexed','0','1','0','-Inf','Inf';'Internal_used2','32','7','LE','unsigned','Multiplexed','0','1','0','-Inf','Inf';'Internal_used3','51','7','LE','unsigned','Multiplexed','0','1','0','-Inf','Inf';'Internal_used4','58','6','LE','unsigned','Multiplexed','0','1','0','-Inf','Inf';'Internal_used5','9','8','LE','unsigned','Multiplexed','1','1','0','-Inf','Inf';'Internal_used6','17','8','LE','unsigned','Multiplexed','1','1','0','-Inf','Inf';'Internal_used7','25','7','LE','unsigned','Multiplexed','1','1','0','-Inf','Inf';'Mode_Signal','0','1','LE','unsigned','Multiplexor','0','1','0','0','1';'RCS','1','7','LE','unsigned','Multiplexed','1','0.2','-15','-15','36';'Range1','1','13','LE','unsigned','Multiplexed','0','0.04','0','0','327.64';'Reserve_3','32','5','LE','unsigned','Multiplexed','1','1','0','-Inf','Inf';'Reserve_4','47','16','LE','unsigned','Multiplexed','1','1','0','-Inf','Inf';'Speed_Radial','39','12','LE','unsigned','Multiplexed','0','0.04','-119.68','-44.12','119.68'}  IDPort=on  TimestampPort=on  ErrorPort=off  RemotePort=off  LengthPort=off  StatusPort=off  ApplyMinMax=off
      settings: DataFormat=CANdb specified signals
  CAN Unpack47 : canmsglib/CAN Unpack  CANdbFile=eWolf_SensorCAN.dbc  MsgList=Radar_RawTarget_Data_046  MsgName=Radar_RawTarget_Data_046  MsgIDType=Standard (11-bit identifier)  MsgIdentifier=1070  MsgLength=8  SignalInfo={'AZ_Winkel','22','10','LE','unsigned','Multiplexed','0','0.16','-81.76','-81.76','81.92';'EL_Angle','37','10','LE','unsigned','Multiplexed','1','0.04','-20.44','-20.44','20.48';'Internal_used','14','8','LE','unsigned','Multiplexed','0','1','0','-Inf','Inf';'Internal_used2','32','7','LE','unsigned','Multiplexed','0','1','0','-Inf','Inf';'Internal_used3','51','7','LE','unsigned','Multiplexed','0','1','0','-Inf','Inf';'Internal_used4','58','6','LE','unsigned','Multiplexed','0','1','0','-Inf','Inf';'Internal_used5','9','8','LE','unsigned','Multiplexed','1','1','0','-Inf','Inf';'Internal_used6','17','8','LE','unsigned','Multiplexed','1','1','0','-Inf','Inf';'Internal_used7','25','7','LE','unsigned','Multiplexed','1','1','0','-Inf','Inf';'Mode_Signal','0','1','LE','unsigned','Multiplexor','0','1','0','0','1';'RCS','1','7','LE','unsigned','Multiplexed','1','0.2','-15','-15','36';'Range1','1','13','LE','unsigned','Multiplexed','0','0.04','0','0','327.64';'Reserve_3','32','5','LE','unsigned','Multiplexed','1','1','0','-Inf','Inf';'Reserve_4','47','16','LE','unsigned','Multiplexed','1','1','0','-Inf','Inf';'Speed_Radial','39','12','LE','unsigned','Multiplexed','0','0.04','-119.68','-44.12','119.68'}  IDPort=on  TimestampPort=on  ErrorPort=off  RemotePort=off  LengthPort=off  StatusPort=off  ApplyMinMax=off
      settings: DataFormat=CANdb specified signals
  CAN Unpack48 : canmsglib/CAN Unpack  CANdbFile=eWolf_SensorCAN.dbc  MsgList=Radar_RawTarget_Data_047  MsgName=Radar_RawTarget_Data_047  MsgIDType=Standard (11-bit identifier)  MsgIdentifier=1071  MsgLength=8  SignalInfo={'AZ_Winkel','22','10','LE','unsigned','Multiplexed','0','0.16','-81.76','-81.76','81.92';'EL_Angle','37','10','LE','unsigned','Multiplexed','1','0.04','-20.44','-20.44','20.48';'Internal_used','14','8','LE','unsigned','Multiplexed','0','1','0','-Inf','Inf';'Internal_used2','32','7','LE','unsigned','Multiplexed','0','1','0','-Inf','Inf';'Internal_used3','51','7','LE','unsigned','Multiplexed','0','1','0','-Inf','Inf';'Internal_used4','58','6','LE','unsigned','Multiplexed','0','1','0','-Inf','Inf';'Internal_used5','9','8','LE','unsigned','Multiplexed','1','1','0','-Inf','Inf';'Internal_used6','17','8','LE','unsigned','Multiplexed','1','1','0','-Inf','Inf';'Internal_used7','25','7','LE','unsigned','Multiplexed','1','1','0','-Inf','Inf';'Mode_Signal','0','1','LE','unsigned','Multiplexor','0','1','0','0','1';'RCS','1','7','LE','unsigned','Multiplexed','1','0.2','-15','-15','36';'Range1','1','13','LE','unsigned','Multiplexed','0','0.04','0','0','327.64';'Reserve_3','32','5','LE','unsigned','Multiplexed','1','1','0','-Inf','Inf';'Reserve_4','47','16','LE','unsigned','Multiplexed','1','1','0','-Inf','Inf';'Speed_Radial','39','12','LE','unsigned','Multiplexed','0','0.04','-119.68','-44.12','119.68'}  IDPort=on  TimestampPort=on  ErrorPort=off  RemotePort=off  LengthPort=off  StatusPort=off  ApplyMinMax=off
      settings: DataFormat=CANdb specified signals
  CAN Unpack49 : canmsglib/CAN Unpack  CANdbFile=eWolf_SensorCAN.dbc  MsgList=Radar_RawTarget_Data_048  MsgName=Radar_RawTarget_Data_048  MsgIDType=Standard (11-bit identifier)  MsgIdentifier=1072  MsgLength=8  SignalInfo={'AZ_Winkel','22','10','LE','unsigned','Multiplexed','0','0.16','-81.76','-81.76','81.92';'EL_Angle','37','10','LE','unsigned','Multiplexed','1','0.04','-20.44','-20.44','20.48';'Internal_used','14','8','LE','unsigned','Multiplexed','0','1','0','-Inf','Inf';'Internal_used2','32','7','LE','unsigned','Multiplexed','0','1','0','-Inf','Inf';'Internal_used3','51','7','LE','unsigned','Multiplexed','0','1','0','-Inf','Inf';'Internal_used4','58','6','LE','unsigned','Multiplexed','0','1','0','-Inf','Inf';'Internal_used5','9','8','LE','unsigned','Multiplexed','1','1','0','-Inf','Inf';'Internal_used6','17','8','LE','unsigned','Multiplexed','1','1','0','-Inf','Inf';'Internal_used7','25','7','LE','unsigned','Multiplexed','1','1','0','-Inf','Inf';'Mode_Signal','0','1','LE','unsigned','Multiplexor','0','1','0','0','1';'RCS','1','7','LE','unsigned','Multiplexed','1','0.2','-15','-15','36';'Range1','1','13','LE','unsigned','Multiplexed','0','0.04','0','0','327.64';'Reserve_3','32','5','LE','unsigned','Multiplexed','1','1','0','-Inf','Inf';'Reserve_4','47','16','LE','unsigned','Multiplexed','1','1','0','-Inf','Inf';'Speed_Radial','39','12','LE','unsigned','Multiplexed','0','0.04','-119.68','-44.12','119.68'}  IDPort=on  TimestampPort=on  ErrorPort=off  RemotePort=off  LengthPort=off  StatusPort=off  ApplyMinMax=off
      settings: DataFormat=CANdb specified signals
  CAN Unpack5 : canmsglib/CAN Unpack  CANdbFile=eWolf_SensorCAN.dbc  MsgList=Radar_RawTarget_Data_004  MsgName=Radar_RawTarget_Data_004  MsgIDType=Standard (11-bit identifier)  MsgIdentifier=1028  MsgLength=8  SignalInfo={'AZ_Winkel','22','10','LE','unsigned','Multiplexed','0','0.16','-81.76','-81.76','81.92';'EL_Angle','37','10','LE','unsigned','Multiplexed','1','0.04','-20.44','-20.44','20.48';'Internal_used','14','8','LE','unsigned','Multiplexed','0','1','0','-Inf','Inf';'Internal_used2','32','7','LE','unsigned','Multiplexed','0','1','0','-Inf','Inf';'Internal_used3','51','7','LE','unsigned','Multiplexed','0','1','0','-Inf','Inf';'Internal_used4','58','6','LE','unsigned','Multiplexed','0','1','0','-Inf','Inf';'Internal_used5','9','8','LE','unsigned','Multiplexed','1','1','0','-Inf','Inf';'Internal_used6','17','8','LE','unsigned','Multiplexed','1','1','0','-Inf','Inf';'Internal_used7','25','7','LE','unsigned','Multiplexed','1','1','0','-Inf','Inf';'Mode_Signal','0','1','LE','unsigned','Multiplexor','0','1','0','0','1';'RCS','1','7','LE','unsigned','Multiplexed','1','0.2','-15','-15','36';'Range1','1','13','LE','unsigned','Multiplexed','0','0.04','0','0','327.64';'Reserve_3','32','5','LE','unsigned','Multiplexed','1','1','0','-Inf','Inf';'Reserve_4','47','16','LE','unsigned','Multiplexed','1','1','0','-Inf','Inf';'Speed_Radial','39','12','LE','unsigned','Multiplexed','0','0.04','-119.68','-44.12','119.68'}  IDPort=on  TimestampPort=on  ErrorPort=off  RemotePort=off  LengthPort=off  StatusPort=off  ApplyMinMax=off
      settings: DataFormat=CANdb specified signals
  CAN Unpack50 : canmsglib/CAN Unpack  CANdbFile=eWolf_SensorCAN.dbc  MsgList=Radar_RawTarget_Data_049  MsgName=Radar_RawTarget_Data_049  MsgIDType=Standard (11-bit identifier)  MsgIdentifier=1073  MsgLength=8  SignalInfo={'AZ_Winkel','22','10','LE','unsigned','Multiplexed','0','0.16','-81.76','-81.76','81.92';'EL_Angle','37','10','LE','unsigned','Multiplexed','1','0.04','-20.44','-20.44','20.48';'Internal_used','14','8','LE','unsigned','Multiplexed','0','1','0','-Inf','Inf';'Internal_used2','32','7','LE','unsigned','Multiplexed','0','1','0','-Inf','Inf';'Internal_used3','51','7','LE','unsigned','Multiplexed','0','1','0','-Inf','Inf';'Internal_used4','58','6','LE','unsigned','Multiplexed','0','1','0','-Inf','Inf';'Internal_used5','9','8','LE','unsigned','Multiplexed','1','1','0','-Inf','Inf';'Internal_used6','17','8','LE','unsigned','Multiplexed','1','1','0','-Inf','Inf';'Internal_used7','25','7','LE','unsigned','Multiplexed','1','1','0','-Inf','Inf';'Mode_Signal','0','1','LE','unsigned','Multiplexor','0','1','0','0','1';'RCS','1','7','LE','unsigned','Multiplexed','1','0.2','-15','-15','36';'Range1','1','13','LE','unsigned','Multiplexed','0','0.04','0','0','327.64';'Reserve_3','32','5','LE','unsigned','Multiplexed','1','1','0','-Inf','Inf';'Reserve_4','47','16','LE','unsigned','Multiplexed','1','1','0','-Inf','Inf';'Speed_Radial','39','12','LE','unsigned','Multiplexed','0','0.04','-119.68','-44.12','119.68'}  IDPort=on  TimestampPort=on  ErrorPort=off  RemotePort=off  LengthPort=off  StatusPort=off  ApplyMinMax=off
      settings: DataFormat=CANdb specified signals
  CAN Unpack51 : canmsglib/CAN Unpack  CANdbFile=eWolf_SensorCAN.dbc  MsgList=Radar_RawTarget_Data_050  MsgName=Radar_RawTarget_Data_050  MsgIDType=Standard (11-bit identifier)  MsgIdentifier=1074  MsgLength=8  SignalInfo={'AZ_Winkel','22','10','LE','unsigned','Multiplexed','0','0.16','-81.76','-81.76','81.92';'EL_Angle','37','10','LE','unsigned','Multiplexed','1','0.04','-20.44','-20.44','20.48';'Internal_used','14','8','LE','unsigned','Multiplexed','0','1','0','-Inf','Inf';'Internal_used2','32','7','LE','unsigned','Multiplexed','0','1','0','-Inf','Inf';'Internal_used3','51','7','LE','unsigned','Multiplexed','0','1','0','-Inf','Inf';'Internal_used4','58','6','LE','unsigned','Multiplexed','0','1','0','-Inf','Inf';'Internal_used5','9','8','LE','unsigned','Multiplexed','1','1','0','-Inf','Inf';'Internal_used6','17','8','LE','unsigned','Multiplexed','1','1','0','-Inf','Inf';'Internal_used7','25','7','LE','unsigned','Multiplexed','1','1','0','-Inf','Inf';'Mode_Signal','0','1','LE','unsigned','Multiplexor','0','1','0','0','1';'RCS','1','7','LE','unsigned','Multiplexed','1','0.2','-15','-15','36';'Range1','1','13','LE','unsigned','Multiplexed','0','0.04','0','0','327.64';'Reserve_3','32','5','LE','unsigned','Multiplexed','1','1','0','-Inf','Inf';'Reserve_4','47','16','LE','unsigned','Multiplexed','1','1','0','-Inf','Inf';'Speed_Radial','39','12','LE','unsigned','Multiplexed','0','0.04','-119.68','-44.12','119.68'}  IDPort=on  TimestampPort=on  ErrorPort=off  RemotePort=off  LengthPort=off  StatusPort=off  ApplyMinMax=off
      settings: DataFormat=CANdb specified signals
  CAN Unpack52 : canmsglib/CAN Unpack  CANdbFile=eWolf_SensorCAN.dbc  MsgList=Radar_RawTarget_Data_051  MsgName=Radar_RawTarget_Data_051  MsgIDType=Standard (11-bit identifier)  MsgIdentifier=1075  MsgLength=8  SignalInfo={'AZ_Winkel','22','10','LE','unsigned','Multiplexed','0','0.16','-81.76','-81.76','81.92';'EL_Angle','37','10','LE','unsigned','Multiplexed','1','0.04','-20.44','-20.44','20.48';'Internal_used','14','8','LE','unsigned','Multiplexed','0','1','0','-Inf','Inf';'Internal_used2','32','7','LE','unsigned','Multiplexed','0','1','0','-Inf','Inf';'Internal_used3','51','7','LE','unsigned','Multiplexed','0','1','0','-Inf','Inf';'Internal_used4','58','6','LE','unsigned','Multiplexed','0','1','0','-Inf','Inf';'Internal_used5','9','8','LE','unsigned','Multiplexed','1','1','0','-Inf','Inf';'Internal_used6','17','8','LE','unsigned','Multiplexed','1','1','0','-Inf','Inf';'Internal_used7','25','7','LE','unsigned','Multiplexed','1','1','0','-Inf','Inf';'Mode_Signal','0','1','LE','unsigned','Multiplexor','0','1','0','0','1';'RCS','1','7','LE','unsigned','Multiplexed','1','0.2','-15','-15','36';'Range1','1','13','LE','unsigned','Multiplexed','0','0.04','0','0','327.64';'Reserve_3','32','5','LE','unsigned','Multiplexed','1','1','0','-Inf','Inf';'Reserve_4','47','16','LE','unsigned','Multiplexed','1','1','0','-Inf','Inf';'Speed_Radial','39','12','LE','unsigned','Multiplexed','0','0.04','-119.68','-44.12','119.68'}  IDPort=on  TimestampPort=on  ErrorPort=off  RemotePort=off  LengthPort=off  StatusPort=off  ApplyMinMax=off
      settings: DataFormat=CANdb specified signals
  CAN Unpack53 : canmsglib/CAN Unpack  CANdbFile=eWolf_SensorCAN.dbc  MsgList=Radar_RawTarget_Data_052  MsgName=Radar_RawTarget_Data_052  MsgIDType=Standard (11-bit identifier)  MsgIdentifier=1076  MsgLength=8  SignalInfo={'AZ_Winkel','22','10','LE','unsigned','Multiplexed','0','0.16','-81.76','-81.76','81.92';'EL_Angle','37','10','LE','unsigned','Multiplexed','1','0.04','-20.44','-20.44','20.48';'Internal_used','14','8','LE','unsigned','Multiplexed','0','1','0','-Inf','Inf';'Internal_used2','32','7','LE','unsigned','Multiplexed','0','1','0','-Inf','Inf';'Internal_used3','51','7','LE','unsigned','Multiplexed','0','1','0','-Inf','Inf';'Internal_used4','58','6','LE','unsigned','Multiplexed','0','1','0','-Inf','Inf';'Internal_used5','9','8','LE','unsigned','Multiplexed','1','1','0','-Inf','Inf';'Internal_used6','17','8','LE','unsigned','Multiplexed','1','1','0','-Inf','Inf';'Internal_used7','25','7','LE','unsigned','Multiplexed','1','1','0','-Inf','Inf';'Mode_Signal','0','1','LE','unsigned','Multiplexor','0','1','0','0','1';'RCS','1','7','LE','unsigned','Multiplexed','1','0.2','-15','-15','36';'Range1','1','13','LE','unsigned','Multiplexed','0','0.04','0','0','327.64';'Reserve_3','32','5','LE','unsigned','Multiplexed','1','1','0','-Inf','Inf';'Reserve_4','47','16','LE','unsigned','Multiplexed','1','1','0','-Inf','Inf';'Speed_Radial','39','12','LE','unsigned','Multiplexed','0','0.04','-119.68','-44.12','119.68'}  IDPort=on  TimestampPort=on  ErrorPort=off  RemotePort=off  LengthPort=off  StatusPort=off  ApplyMinMax=off
      settings: DataFormat=CANdb specified signals
  CAN Unpack54 : canmsglib/CAN Unpack  CANdbFile=eWolf_SensorCAN.dbc  MsgList=Radar_RawTarget_Data_053  MsgName=Radar_RawTarget_Data_053  MsgIDType=Standard (11-bit identifier)  MsgIdentifier=1077  MsgLength=8  SignalInfo={'AZ_Winkel','22','10','LE','unsigned','Multiplexed','0','0.16','-81.76','-81.76','81.92';'EL_Angle','37','10','LE','unsigned','Multiplexed','1','0.04','-20.44','-20.44','20.48';'Internal_used','14','8','LE','unsigned','Multiplexed','0','1','0','-Inf','Inf';'Internal_used2','32','7','LE','unsigned','Multiplexed','0','1','0','-Inf','Inf';'Internal_used3','51','7','LE','unsigned','Multiplexed','0','1','0','-Inf','Inf';'Internal_used4','58','6','LE','unsigned','Multiplexed','0','1','0','-Inf','Inf';'Internal_used5','9','8','LE','unsigned','Multiplexed','1','1','0','-Inf','Inf';'Internal_used6','17','8','LE','unsigned','Multiplexed','1','1','0','-Inf','Inf';'Internal_used7','25','7','LE','unsigned','Multiplexed','1','1','0','-Inf','Inf';'Mode_Signal','0','1','LE','unsigned','Multiplexor','0','1','0','0','1';'RCS','1','7','LE','unsigned','Multiplexed','1','0.2','-15','-15','36';'Range1','1','13','LE','unsigned','Multiplexed','0','0.04','0','0','327.64';'Reserve_3','32','5','LE','unsigned','Multiplexed','1','1','0','-Inf','Inf';'Reserve_4','47','16','LE','unsigned','Multiplexed','1','1','0','-Inf','Inf';'Speed_Radial','39','12','LE','unsigned','Multiplexed','0','0.04','-119.68','-44.12','119.68'}  IDPort=on  TimestampPort=on  ErrorPort=off  RemotePort=off  LengthPort=off  StatusPort=off  ApplyMinMax=off
      settings: DataFormat=CANdb specified signals
  CAN Unpack55 : canmsglib/CAN Unpack  CANdbFile=eWolf_SensorCAN.dbc  MsgList=Radar_RawTarget_Data_054  MsgName=Radar_RawTarget_Data_054  MsgIDType=Standard (11-bit identifier)  MsgIdentifier=1078  MsgLength=8  SignalInfo={'AZ_Winkel','22','10','LE','unsigned','Multiplexed','0','0.16','-81.76','-81.76','81.92';'EL_Angle','37','10','LE','unsigned','Multiplexed','1','0.04','-20.44','-20.44','20.48';'Internal_used','14','8','LE','unsigned','Multiplexed','0','1','0','-Inf','Inf';'Internal_used2','32','7','LE','unsigned','Multiplexed','0','1','0','-Inf','Inf';'Internal_used3','51','7','LE','unsigned','Multiplexed','0','1','0','-Inf','Inf';'Internal_used4','58','6','LE','unsigned','Multiplexed','0','1','0','-Inf','Inf';'Internal_used5','9','8','LE','unsigned','Multiplexed','1','1','0','-Inf','Inf';'Internal_used6','17','8','LE','unsigned','Multiplexed','1','1','0','-Inf','Inf';'Internal_used7','25','7','LE','unsigned','Multiplexed','1','1','0','-Inf','Inf';'Mode_Signal','0','1','LE','unsigned','Multiplexor','0','1','0','0','1';'RCS','1','7','LE','unsigned','Multiplexed','1','0.2','-15','-15','36';'Range1','1','13','LE','unsigned','Multiplexed','0','0.04','0','0','327.64';'Reserve_3','32','5','LE','unsigned','Multiplexed','1','1','0','-Inf','Inf';'Reserve_4','47','16','LE','unsigned','Multiplexed','1','1','0','-Inf','Inf';'Speed_Radial','39','12','LE','unsigned','Multiplexed','0','0.04','-119.68','-44.12','119.68'}  IDPort=on  TimestampPort=on  ErrorPort=off  RemotePort=off  LengthPort=off  StatusPort=off  ApplyMinMax=off
      settings: DataFormat=CANdb specified signals
  CAN Unpack56 : canmsglib/CAN Unpack  CANdbFile=eWolf_SensorCAN.dbc  MsgList=Radar_RawTarget_Data_055  MsgName=Radar_RawTarget_Data_055  MsgIDType=Standard (11-bit identifier)  MsgIdentifier=1079  MsgLength=8  SignalInfo={'AZ_Winkel','22','10','LE','unsigned','Multiplexed','0','0.16','-81.76','-81.76','81.92';'EL_Angle','37','10','LE','unsigned','Multiplexed','1','0.04','-20.44','-20.44','20.48';'Internal_used','14','8','LE','unsigned','Multiplexed','0','1','0','-Inf','Inf';'Internal_used2','32','7','LE','unsigned','Multiplexed','0','1','0','-Inf','Inf';'Internal_used3','51','7','LE','unsigned','Multiplexed','0','1','0','-Inf','Inf';'Internal_used4','58','6','LE','unsigned','Multiplexed','0','1','0','-Inf','Inf';'Internal_used5','9','8','LE','unsigned','Multiplexed','1','1','0','-Inf','Inf';'Internal_used6','17','8','LE','unsigned','Multiplexed','1','1','0','-Inf','Inf';'Internal_used7','25','7','LE','unsigned','Multiplexed','1','1','0','-Inf','Inf';'Mode_Signal','0','1','LE','unsigned','Multiplexor','0','1','0','0','1';'RCS','1','7','LE','unsigned','Multiplexed','1','0.2','-15','-15','36';'Range1','1','13','LE','unsigned','Multiplexed','0','0.04','0','0','327.64';'Reserve_3','32','5','LE','unsigned','Multiplexed','1','1','0','-Inf','Inf';'Reserve_4','47','16','LE','unsigned','Multiplexed','1','1','0','-Inf','Inf';'Speed_Radial','39','12','LE','unsigned','Multiplexed','0','0.04','-119.68','-44.12','119.68'}  IDPort=on  TimestampPort=on  ErrorPort=off  RemotePort=off  LengthPort=off  StatusPort=off  ApplyMinMax=off
      settings: DataFormat=CANdb specified signals
  CAN Unpack57 : canmsglib/CAN Unpack  CANdbFile=eWolf_SensorCAN.dbc  MsgList=Radar_RawTarget_Data_056  MsgName=Radar_RawTarget_Data_056  MsgIDType=Standard (11-bit identifier)  MsgIdentifier=1080  MsgLength=8  SignalInfo={'AZ_Winkel','22','10','LE','unsigned','Multiplexed','0','0.16','-81.76','-81.76','81.92';'EL_Angle','37','10','LE','unsigned','Multiplexed','1','0.04','-20.44','-20.44','20.48';'Internal_used','14','8','LE','unsigned','Multiplexed','0','1','0','-Inf','Inf';'Internal_used2','32','7','LE','unsigned','Multiplexed','0','1','0','-Inf','Inf';'Internal_used3','51','7','LE','unsigned','Multiplexed','0','1','0','-Inf','Inf';'Internal_used4','58','6','LE','unsigned','Multiplexed','0','1','0','-Inf','Inf';'Internal_used5','9','8','LE','unsigned','Multiplexed','1','1','0','-Inf','Inf';'Internal_used6','17','8','LE','unsigned','Multiplexed','1','1','0','-Inf','Inf';'Internal_used7','25','7','LE','unsigned','Multiplexed','1','1','0','-Inf','Inf';'Mode_Signal','0','1','LE','unsigned','Multiplexor','0','1','0','0','1';'RCS','1','7','LE','unsigned','Multiplexed','1','0.2','-15','-15','36';'Range1','1','13','LE','unsigned','Multiplexed','0','0.04','0','0','327.64';'Reserve_3','32','5','LE','unsigned','Multiplexed','1','1','0','-Inf','Inf';'Reserve_4','47','16','LE','unsigned','Multiplexed','1','1','0','-Inf','Inf';'Speed_Radial','39','12','LE','unsigned','Multiplexed','0','0.04','-119.68','-44.12','119.68'}  IDPort=on  TimestampPort=on  ErrorPort=off  RemotePort=off  LengthPort=off  StatusPort=off  ApplyMinMax=off
      settings: DataFormat=CANdb specified signals
  CAN Unpack58 : canmsglib/CAN Unpack  CANdbFile=eWolf_SensorCAN.dbc  MsgList=Radar_RawTarget_Data_057  MsgName=Radar_RawTarget_Data_057  MsgIDType=Standard (11-bit identifier)  MsgIdentifier=1081  MsgLength=8  SignalInfo={'AZ_Winkel','22','10','LE','unsigned','Multiplexed','0','0.16','-81.76','-81.76','81.92';'EL_Angle','37','10','LE','unsigned','Multiplexed','1','0.04','-20.44','-20.44','20.48';'Internal_used','14','8','LE','unsigned','Multiplexed','0','1','0','-Inf','Inf';'Internal_used2','32','7','LE','unsigned','Multiplexed','0','1','0','-Inf','Inf';'Internal_used3','51','7','LE','unsigned','Multiplexed','0','1','0','-Inf','Inf';'Internal_used4','58','6','LE','unsigned','Multiplexed','0','1','0','-Inf','Inf';'Internal_used5','9','8','LE','unsigned','Multiplexed','1','1','0','-Inf','Inf';'Internal_used6','17','8','LE','unsigned','Multiplexed','1','1','0','-Inf','Inf';'Internal_used7','25','7','LE','unsigned','Multiplexed','1','1','0','-Inf','Inf';'Mode_Signal','0','1','LE','unsigned','Multiplexor','0','1','0','0','1';'RCS','1','7','LE','unsigned','Multiplexed','1','0.2','-15','-15','36';'Range1','1','13','LE','unsigned','Multiplexed','0','0.04','0','0','327.64';'Reserve_3','32','5','LE','unsigned','Multiplexed','1','1','0','-Inf','Inf';'Reserve_4','47','16','LE','unsigned','Multiplexed','1','1','0','-Inf','Inf';'Speed_Radial','39','12','LE','unsigned','Multiplexed','0','0.04','-119.68','-44.12','119.68'}  IDPort=on  TimestampPort=on  ErrorPort=off  RemotePort=off  LengthPort=off  StatusPort=off  ApplyMinMax=off
      settings: DataFormat=CANdb specified signals
  CAN Unpack59 : canmsglib/CAN Unpack  CANdbFile=eWolf_SensorCAN.dbc  MsgList=Radar_RawTarget_Data_058  MsgName=Radar_RawTarget_Data_058  MsgIDType=Standard (11-bit identifier)  MsgIdentifier=1082  MsgLength=8  SignalInfo={'AZ_Winkel','22','10','LE','unsigned','Multiplexed','0','0.16','-81.76','-81.76','81.92';'EL_Angle','37','10','LE','unsigned','Multiplexed','1','0.04','-20.44','-20.44','20.48';'Internal_used','14','8','LE','unsigned','Multiplexed','0','1','0','-Inf','Inf';'Internal_used2','32','7','LE','unsigned','Multiplexed','0','1','0','-Inf','Inf';'Internal_used3','51','7','LE','unsigned','Multiplexed','0','1','0','-Inf','Inf';'Internal_used4','58','6','LE','unsigned','Multiplexed','0','1','0','-Inf','Inf';'Internal_used5','9','8','LE','unsigned','Multiplexed','1','1','0','-Inf','Inf';'Internal_used6','17','8','LE','unsigned','Multiplexed','1','1','0','-Inf','Inf';'Internal_used7','25','7','LE','unsigned','Multiplexed','1','1','0','-Inf','Inf';'Mode_Signal','0','1','LE','unsigned','Multiplexor','0','1','0','0','1';'RCS','1','7','LE','unsigned','Multiplexed','1','0.2','-15','-15','36';'Range1','1','13','LE','unsigned','Multiplexed','0','0.04','0','0','327.64';'Reserve_3','32','5','LE','unsigned','Multiplexed','1','1','0','-Inf','Inf';'Reserve_4','47','16','LE','unsigned','Multiplexed','1','1','0','-Inf','Inf';'Speed_Radial','39','12','LE','unsigned','Multiplexed','0','0.04','-119.68','-44.12','119.68'}  IDPort=on  TimestampPort=on  ErrorPort=off  RemotePort=off  LengthPort=off  StatusPort=off  ApplyMinMax=off
      settings: DataFormat=CANdb specified signals
  CAN Unpack6 : canmsglib/CAN Unpack  CANdbFile=eWolf_SensorCAN.dbc  MsgList=Radar_RawTarget_Data_005  MsgName=Radar_RawTarget_Data_005  MsgIDType=Standard (11-bit identifier)  MsgIdentifier=1029  MsgLength=8  SignalInfo={'AZ_Winkel','22','10','LE','unsigned','Multiplexed','0','0.16','-81.76','-81.76','81.92';'EL_Angle','37','10','LE','unsigned','Multiplexed','1','0.04','-20.44','-20.44','20.48';'Internal_used','14','8','LE','unsigned','Multiplexed','0','1','0','-Inf','Inf';'Internal_used2','32','7','LE','unsigned','Multiplexed','0','1','0','-Inf','Inf';'Internal_used3','51','7','LE','unsigned','Multiplexed','0','1','0','-Inf','Inf';'Internal_used4','58','6','LE','unsigned','Multiplexed','0','1','0','-Inf','Inf';'Internal_used5','9','8','LE','unsigned','Multiplexed','1','1','0','-Inf','Inf';'Internal_used6','17','8','LE','unsigned','Multiplexed','1','1','0','-Inf','Inf';'Internal_used7','25','7','LE','unsigned','Multiplexed','1','1','0','-Inf','Inf';'Mode_Signal','0','1','LE','unsigned','Multiplexor','0','1','0','0','1';'RCS','1','7','LE','unsigned','Multiplexed','1','0.2','-15','-15','36';'Range1','1','13','LE','unsigned','Multiplexed','0','0.04','0','0','327.64';'Reserve_3','32','5','LE','unsigned','Multiplexed','1','1','0','-Inf','Inf';'Reserve_4','47','16','LE','unsigned','Multiplexed','1','1','0','-Inf','Inf';'Speed_Radial','39','12','LE','unsigned','Multiplexed','0','0.04','-119.68','-44.12','119.68'}  IDPort=on  TimestampPort=on  ErrorPort=off  RemotePort=off  LengthPort=off  StatusPort=off  ApplyMinMax=off
      settings: DataFormat=CANdb specified signals
  CAN Unpack60 : canmsglib/CAN Unpack  CANdbFile=eWolf_SensorCAN.dbc  MsgList=Radar_RawTarget_Data_059  MsgName=Radar_RawTarget_Data_059  MsgIDType=Standard (11-bit identifier)  MsgIdentifier=1083  MsgLength=8  SignalInfo={'AZ_Winkel','22','10','LE','unsigned','Multiplexed','0','0.16','-81.76','-81.76','81.92';'EL_Angle','37','10','LE','unsigned','Multiplexed','1','0.04','-20.44','-20.44','20.48';'Internal_used','14','8','LE','unsigned','Multiplexed','0','1','0','-Inf','Inf';'Internal_used2','32','7','LE','unsigned','Multiplexed','0','1','0','-Inf','Inf';'Internal_used3','51','7','LE','unsigned','Multiplexed','0','1','0','-Inf','Inf';'Internal_used4','58','6','LE','unsigned','Multiplexed','0','1','0','-Inf','Inf';'Internal_used5','9','8','LE','unsigned','Multiplexed','1','1','0','-Inf','Inf';'Internal_used6','17','8','LE','unsigned','Multiplexed','1','1','0','-Inf','Inf';'Internal_used7','25','7','LE','unsigned','Multiplexed','1','1','0','-Inf','Inf';'Mode_Signal','0','1','LE','unsigned','Multiplexor','0','1','0','0','1';'RCS','1','7','LE','unsigned','Multiplexed','1','0.2','-15','-15','36';'Range1','1','13','LE','unsigned','Multiplexed','0','0.04','0','0','327.64';'Reserve_3','32','5','LE','unsigned','Multiplexed','1','1','0','-Inf','Inf';'Reserve_4','47','16','LE','unsigned','Multiplexed','1','1','0','-Inf','Inf';'Speed_Radial','39','12','LE','unsigned','Multiplexed','0','0.04','-119.68','-44.12','119.68'}  IDPort=on  TimestampPort=on  ErrorPort=off  RemotePort=off  LengthPort=off  StatusPort=off  ApplyMinMax=off
      settings: DataFormat=CANdb specified signals
